simulink model "mdl_foc_platform"  (R2023a)
settings: configuration reference "cfg_FocCodeGeneration_v04" (kept outside this file)
undefined symbols (not defined in the file): Cdbl_nMechSpdPeakVal, cstPermMagTempCoef, cstPolePairNum, cstRefTemp, Gu16_rCtlBrdVltgADCRat_C, Gu16_rGDVltgADCRat_C, Gu16_rPhCurrADCRat_C, Gu16_rSplyVltgADCRat_C, Gu16_tMotoTemp_CUR_ADMotoTempADC_X, Gu16_tPCBTemp_CUR_ADPCBTempADC_X, Gu16_tPwrTubTemp_CUR_ADPwrTubTempADC_X, Gu8_tMotoTemp_CUR, Gu8_tPCBTemp_CUR, Gu8_tPwrTubTemp_CUR, parAmbPermMagFlux, parDirIndc, parPolePairNum, parQdrtIndc
libraries: lib_conversion x10, eeTransforms x1, simulink x1, lib_park_transform x1
(part 1 of 2)
settings Model: DataDictionary=dd_platform_parameter.sldd  EnableAccessToBaseWorkspace=off  PauseTimes=0.1  Creator=WEIFU_YuanXiaoqiang  LastModifiedBy=xiaoqiang.yuan
settings ConfigSetRef: SourceName=cfg_FocCodeGeneration_v04

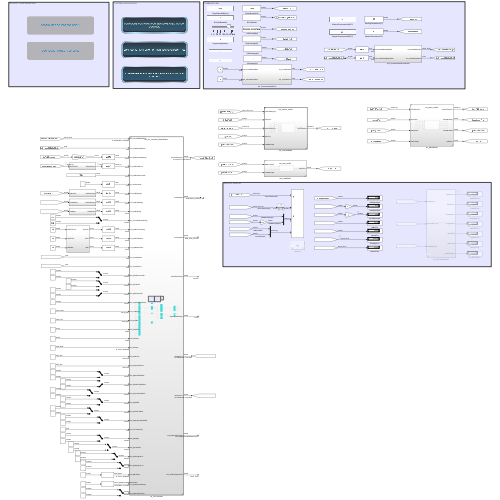
[thumbnail: Simulink's stored preview of the top-level diagram]
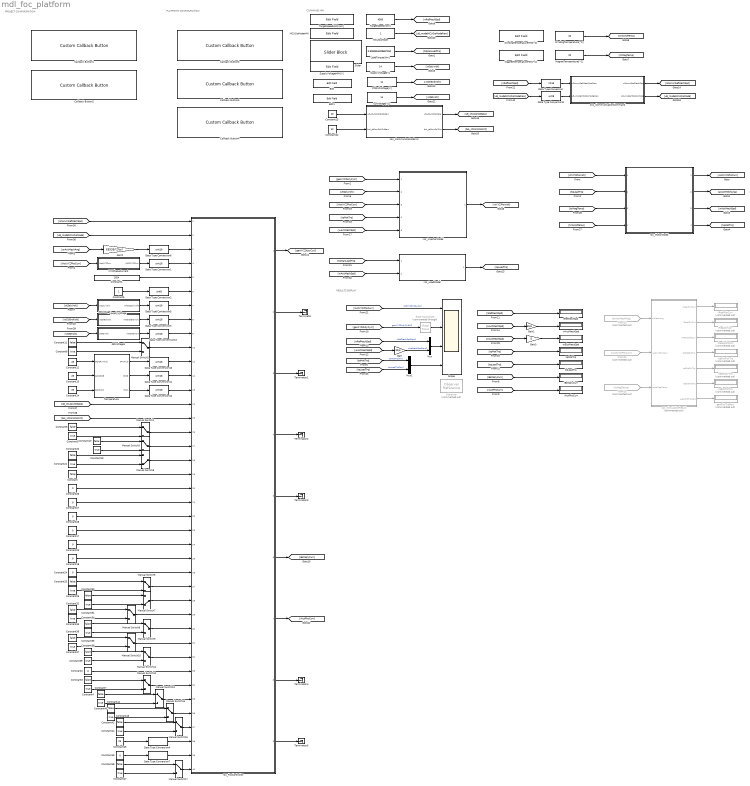
== system mdl_foc_platform ==
  note: PROJECT CONFIGURATION
  note: COMMAND HMI
  note: PLATFORM CONFIGURATION
  note: RESULTS DISPLAY
  Callback Button1 : CustomCallbackButton  Description=BYD 48V Project  Configuration="{\"components\":[{\"name\":\"BackgroundImageComponent\",\"settings\":{\"image\":{\"size\":[0,0],\"src\":\"default\",\"srcOrientation\":\"horizontal\"},\"position\":[0,0,1,1],\"scaleMode\":\"0\"}},{\"name\":\"ButtonStateComponent\",\"settings\":{\"buttonType\":\"momentary\",\"clickFcn\":\"\\nproj = simulinkproject;\\nproj_dir = proj.RootFolder;\\n% configure GEELY\\n%%AST \\nopen_system([proj_dir,'\\\\referenced_model\\\\ASW_AST\\\\ASW_AST.slx']);\\nmodel_path = 'ASW_AST';\\nset_param([model_path,'\\/AST_SlwTask\\/vrs_SysSTM'],...\\n    'LabelModeActiveChoice','GEELY_PROJECT');\\nsave_system([proj_dir,'\\\\referenced_model\\\\ASW_AST\\\\ASW_AST.slx'],'SaveDirtyReferencedModels',true);\\nclose_system([proj_dir,'\\\\referenced_model\\\\ASW_AST\\\\ASW_AST.slx']);\\n\\n%%OBD \\nopen_system([proj_dir,'\\\\referenced_model\\\\ASW_OBD\\\\ASW_OBD.slx']);\\nmodel_path = 'ASW_OBD';\\nset_param([model_path,'\\/OBD_SlwTask\\/rss_ComFaltDia\\/sss_ComFalt\\/ens_HysDeb'],...\\n    'LabelModeActiveChoice','GEELY_PROJECT');\\nset_param([model_path,'\\/OBD_SlwTask\\/rss_FaltResp\\/sss_FaltRespDefd\\/sss_FaltMechSpdRespDefd\\/sss_Else\\/sss_ComFaltMechSpdRespDefd'],...\\n    'LabelModeActiveChoice','GEELY_PROJECT');\\nset_param([model_path,'\\/OBD_SlwTask\\/vrs_FaltEnFlgConf\\/rss_FaltEnFlgConfSenl\\/sss_FaltPrioJudg\\/sss_Else'],...\\n    'LabelModeActiveChoice','GEELY_PROJECT');\\nset_param([model_path,'\\/OBD_SlwTask\\/rss_FaltInfoMng\\/vrs_DSMSaveInfo'],...\\n    'LabelModeActiveChoice','DSMSaveInfoNoNeed');\\nset_param([model_path,'\\/OBD_SlwTask\\/rss_GDVltgLoLvl1Dia\\/sss_GDVltgLoLvl1\\/ens_Deb'],...\\n    'LabelModeActiveChoice','GEELY_PROJECT');\\nset_param([model_path,'\\/OBD_SlwTask\\/rss_GDVltgHiLvl1Dia\\/sss_GDVltgHiLvl1\\/ens_Deb'],...\\n    'LabelModeActiveChoice','GEELY_PROJECT');\\nsave_system([proj_dir,'\\\\referenced_model\\\\ASW_OBD\\\\ASW_OBD.slx'],'SaveDirtyReferencedModels',true);\\nclose_system([proj_dir,'\\\\referenced_model\\\\ASW_OBD\\\\ASW_OBD.slx']);\\n\",\"image\":{\"size\":[180,45],\"srcOrientation\":\"Right\"},\"onValue\":1,\"position\":[0,0,1,1],\"pressDelay\":\"500\",\"pressFcn\":\"\",\"repeatInterval\":\"0\",\"states\":[{\"horizontalAlignment\":\"center\",\"image\":{\"position\":[0.04444444444444445,0.005555555555555536,0.9888888888888889,0.9111111111111111],\"size\":[0.9888888888888889,0.9111111111111111],\"src\":\"data:image\\/svg+xml;base64,PHN2ZyB4bWxucz0iaHR0cDovL3d3dy53My5vcmcvMjAwMC9zdmciIHhtbG5zOnhsaW5rPSJodHRwOi8vd3d3LnczLm9yZy8xOTk5L3hsaW5rIiB2aWV3Qm94PSIwIDAgMTc3LjI1IDQwLjg4Ij48ZGVmcz48c3R5bGU+LmNscy0xe2ZpbGw6dXJsKCNyYWRpYWwtZ3JhZGllbnQpO30uY2xzLTJ7ZmlsbDp1cmwoI2xpbmVhci1ncmFkaWVudCk7fS5jbHMtM3tmaWxsOnVybCgjbGluZWFyLWdyYWRpZW50LTIpO308L3N0eWxlPjxyYWRpYWxHcmFkaWVudCBpZD0icmFkaWFsLWdyYWRpZW50IiBjeD0iOTAuMDkiIGN5PSIyMi42NiIgcj0i ...(+2212 chars)\",\"srcOrientation\":\"Right\"},\"label\":{\"color\":[0,0.4470588235294118,0.7411764705882353],\"icon\":{\"size\":[0,0],\"src\":[],\"srcOrientation\":\"Right\"},\"iconPlacement\":\"left\",\"opacity\":1,\"show\":true,\"text\":{\"content\":\"CONFIGURE PROJECT FOR GEELY\",\"font\":\"Helvetica\",\"fontSize\":4.2}},\"labelOffset\":[0,0],\"verticalAlignment\":\"middle\"},{\"horizontalAlignment\":\"center\",\"image\":{\"position\":[0.04444444444444445,0.005555555555555536,0.9888888888888889,0.9111111111111111],\"size\":[0.9888888888888889,0.9111111111111111],\"src\":\"data:image\\/svg+xml;base64,PHN2ZyB4bWxucz0iaHR0cDovL3d3dy53My5vcmcvMjAwMC9zdmciIHhtbG5zOnhsaW5rPSJodHRwOi8vd3d3LnczLm9yZy8xOTk5L3hsaW5rIiB2aWV3Qm94PSIwIDAgMTc3LjI1IDQwLjg4Ij48ZGVmcz48c3R5bGU+LmNscy0xe2ZpbGw6dXJsKCNyYWRpYWwtZ3JhZGllbnQpO30uY2xzLTJ7ZmlsbDp1cmwoI2xpbmVhci1ncmFkaWVudCk7fS5jbHMtM3tmaWxsOnVybCgjbGluZWFyLWdyYWRpZW50LTIpO308L3N0eWxlPjxyYWRpYWxHcmFkaWVudCBpZD0icmFkaWFsLWdyYWRpZW50IiBjeD0iOTAuMDkiIGN5PSIyMi42NiIgcj0i ...(+2216 chars)\",\"srcOrientation\":\"Right\"},\"label\":{\"color\":[1,1,0.78,1],\"icon\":{\"size\":[0,0],\"src\":[],\"srcOrientation\":\"Right\"},\"iconPlacement\":\"left\",\"opacity\":1,\"show\":true,\"text\":{\"content\":\"CONFIGURE PROJECT FOR GEELY\",\"font\":\"Helvetica\",\"fontSize\":4.2}},\"labelOffset\":[0.025,0],\"verticalAlignment\":\"middle\"},{\"horizontalAlignment\":\"center\",\"image\":{\"position\":[0.04444444444444445,0.005555555555555536,0.9888888888888889,0.9111111111111111],\"size\":[0.9888888888888889,0.9111111111111111],\"src\":\"data:image\\/svg+xml;base64,PHN2ZyB4bWxucz0iaHR0cDovL3d3dy53My5vcmcvMjAwMC9zdmciIHhtbG5zOnhsaW5rPSJodHRwOi8vd3d3LnczLm9yZy8xOTk5L3hsaW5rIiB2aWV3Qm94PSIwIDAgMTc3LjI1IDQwLjg4Ij48ZGVmcz48c3R5bGU+LmNscy0xe2ZpbGw6dXJsKCNyYWRpYWwtZ3JhZGllbnQpO30uY2xzLTJ7ZmlsbDp1cmwoI2xpbmVhci1ncmFkaWVudCk7fS5jbHMtM3tmaWxsOnVybCgjbGluZWFyLWdyYWRpZW50LTIpO308L3N0eWxlPjxyYWRpYWxHcmFkaWVudCBpZD0icmFkaWFsLWdyYWRpZW50IiBjeD0iOTAuMDkiIGN5PSIyMi42NiIgcj0i ...(+2212 chars)\",\"srcOrientation\":\"Right\"},\"label\":{\"color\":[1,1,0.78,1],\"icon\":{\"size\":[0,0],\"src\":[],\"srcOrientation\":\"Right\"},\"iconPlacement\":\"left\",\"opacity\":1,\"show\":true,\"text\":{\"content\":\"CONFIGURE PROJECT FOR GEELY\",\"font\":\"Helvetica\",\"fontSize\":4.2}},\"labelOffset\":[0,0],\"verticalAlignment\":\"middle\"},{\"horizontalAlignment\":\"center\",\"image\":{\"position\":[0.04444444444444445,0.005555555555555536,0.9888888888888889,0.9111111111111111],\"size\":[0.9888888888888889,0.9111111111111111],\"src\":\"data:image\\/svg+xml;base64,PHN2ZyB4bWxucz0iaHR0cDovL3d3dy53My5vcmcvMjAwMC9zdmciIHhtbG5zOnhsaW5rPSJodHRwOi8vd3d3LnczLm9yZy8xOTk5L3hsaW5rIiB2aWV3Qm94PSIwIDAgMTc3LjI1IDQwLjg4Ij48ZGVmcz48c3R5bGU+LmNscy0xe2ZpbGw6dXJsKCNyYWRpYWwtZ3JhZGllbnQpO30uY2xzLTJ7ZmlsbDp1cmwoI2xpbmVhci1ncmFkaWVudCk7fS5jbHMtM3tmaWxsOnVybCgjbGluZWFyLWdyYWRpZW50LTIpO308L3N0eWxlPjxyYWRpYWxHcmFkaWVudCBpZD0icmFkaWFsLWdyYWRpZW50IiBjeD0iOTAuMDkiIGN5PSIyMi42NiIgcj0i ...(+2216 chars)\",\"srcOrientation\":\"Right\"},\"label\":{\"color\":[1,1,0.78,1],\"icon\":{\"size\":[0,0],\"src\":[],\"srcOrientation\":\"Right\"},\"iconPlacement\":\"left\",\"opacity\":1,\"show\":true,\"text\":{\"content\":\"CONFIGURE PROJECT FOR GEELY\",\"font\":\"Helvetica\",\"fontSize\":4.2}},\"labelOffset\":[0.025,0],\"verticalAlignment\":\"middle\"}]}},{\"name\":\"ForegroundImageComponent\",\"settings\":{\"image\":{\"size\":[0,0],\"src\":\"default\",\"srcOrientation\":\"horizontal\"},\"isForeground\":1,\"position\":[0,0,1,1],\"scaleMode\":\"0\"}}],\"settings\":{\"BindingType\":\"param\",\"aspectRatio\":3.7777777777777777,\"backgroundColor\":[255,255,255,\"1\"],\"backgroundOffset\":0.5,\"backgroundOpacity\":1,\"fixedAspectRatio\":\"off\",\"foregroundColor\":[252,252,196],\"showBackgroundColor\":false,\"variant\":\"callback\",\"version\":\"R2022b\"},\"type\":\"Button\"}"  CustomBackgroundColor="{\"color\":[0.6509803921568628,0.6509803921568628,0.6509803921568628],\"show\":true}"
  Callback Button2 : CustomCallbackButton  Description=BYD 48V Project  Configuration="{\"components\":[{\"name\":\"BackgroundImageComponent\",\"settings\":{\"image\":{\"size\":[0,0],\"src\":\"default\",\"srcOrientation\":\"horizontal\"},\"position\":[0,0,1,1],\"scaleMode\":\"0\"}},{\"name\":\"ButtonStateComponent\",\"settings\":{\"buttonType\":\"momentary\",\"clickFcn\":\"\\nproj = simulinkproject;\\nproj_dir = proj.RootFolder;\\n% configure CRRC\\n%%AST \\nopen_system([proj_dir,'\\\\referenced_model\\\\ASW_AST\\\\ASW_AST.slx']);\\nmodel_path = 'ASW_AST';\\nset_param([model_path,'\\/AST_SlwTask\\/vrs_SysSTM'],...\\n    'LabelModeActiveChoice','CRRC_PROJECT');\\nsave_system([proj_dir,'\\\\referenced_model\\\\ASW_AST\\\\ASW_AST.slx'],'SaveDirtyReferencedModels',true);\\nclose_system([proj_dir,'\\\\referenced_model\\\\ASW_AST\\\\ASW_AST.slx']);\\n\\n%%OBD \\nopen_system([proj_dir,'\\\\referenced_model\\\\ASW_OBD\\\\ASW_OBD.slx']);\\nmodel_path = 'ASW_OBD';\\nset_param([model_path,'\\/OBD_SlwTask\\/rss_ComFaltDia\\/sss_ComFalt\\/ens_HysDeb'],...\\n    'LabelModeActiveChoice','CRRC_PROJECT');\\nset_param([model_path,'\\/OBD_SlwTask\\/rss_FaltResp\\/sss_FaltRespDefd\\/sss_FaltMechSpdRespDefd\\/sss_Else\\/sss_ComFaltMechSpdRespDefd'],...\\n    'LabelModeActiveChoice','CRRC_PROJECT');\\nset_param([model_path,'\\/OBD_SlwTask\\/vrs_FaltEnFlgConf\\/rss_FaltEnFlgConfSenl\\/sss_FaltPrioJudg\\/sss_Else'],...\\n    'LabelModeActiveChoice','CRRC_PROJECT');\\nset_param([model_path,'\\/OBD_SlwTask\\/rss_FaltInfoMng\\/vrs_DSMSaveInfo'],...\\n    'LabelModeActiveChoice','DSMSaveInfoNeed');\\nset_param([model_path,'\\/OBD_SlwTask\\/rss_GDVltgLoLvl1Dia\\/sss_GDVltgLoLvl1\\/ens_Deb'],...\\n    'LabelModeActiveChoice','CRRC_PROJECT');\\nset_param([model_path,'\\/OBD_SlwTask\\/rss_GDVltgHiLvl1Dia\\/sss_GDVltgHiLvl1\\/ens_Deb'],...\\n    'LabelModeActiveChoice','CRRC_PROJECT');\\nsave_system([proj_dir,'\\\\referenced_model\\\\ASW_OBD\\\\ASW_OBD.slx'],'SaveDirtyReferencedModels',true);\\nclose_system([proj_dir,'\\\\referenced_model\\\\ASW_OBD\\\\ASW_OBD.slx']);\\n\",\"image\":{\"size\":[180,45],\"srcOrientation\":\"Right\"},\"onValue\":1,\"position\":[0,0,1,1],\"pressDelay\":\"500\",\"pressFcn\":\"\",\"repeatInterval\":\"0\",\"states\":[{\"horizontalAlignment\":\"center\",\"image\":{\"position\":[0.04444444444444445,0.005555555555555536,0.9888888888888889,0.9111111111111111],\"size\":[0.9888888888888889,0.9111111111111111],\"src\":\"data:image\\/svg+xml;base64,PHN2ZyB4bWxucz0iaHR0cDovL3d3dy53My5vcmcvMjAwMC9zdmciIHhtbG5zOnhsaW5rPSJodHRwOi8vd3d3LnczLm9yZy8xOTk5L3hsaW5rIiB2aWV3Qm94PSIwIDAgMTc3LjI1IDQwLjg4Ij48ZGVmcz48c3R5bGU+LmNscy0xe2ZpbGw6dXJsKCNyYWRpYWwtZ3JhZGllbnQpO30uY2xzLTJ7ZmlsbDp1cmwoI2xpbmVhci1ncmFkaWVudCk7fS5jbHMtM3tmaWxsOnVybCgjbGluZWFyLWdyYWRpZW50LTIpO308L3N0eWxlPjxyYWRpYWxHcmFkaWVudCBpZD0icmFkaWFsLWdyYWRpZW50IiBjeD0iOTAuMDkiIGN5PSIyMi42NiIgcj0i ...(+2212 chars)\",\"srcOrientation\":\"Right\"},\"label\":{\"color\":[0,0.4470588235294118,0.7411764705882353],\"icon\":{\"size\":[0,0],\"src\":[],\"srcOrientation\":\"Right\"},\"iconPlacement\":\"left\",\"opacity\":1,\"show\":true,\"text\":{\"content\":\"CONFIGURE PROJECT FOR CRRC\",\"font\":\"Helvetica\",\"fontSize\":4.2}},\"labelOffset\":[0,0],\"verticalAlignment\":\"middle\"},{\"horizontalAlignment\":\"center\",\"image\":{\"position\":[0.04444444444444445,0.005555555555555536,0.9888888888888889,0.9111111111111111],\"size\":[0.9888888888888889,0.9111111111111111],\"src\":\"data:image\\/svg+xml;base64,PHN2ZyB4bWxucz0iaHR0cDovL3d3dy53My5vcmcvMjAwMC9zdmciIHhtbG5zOnhsaW5rPSJodHRwOi8vd3d3LnczLm9yZy8xOTk5L3hsaW5rIiB2aWV3Qm94PSIwIDAgMTc3LjI1IDQwLjg4Ij48ZGVmcz48c3R5bGU+LmNscy0xe2ZpbGw6dXJsKCNyYWRpYWwtZ3JhZGllbnQpO30uY2xzLTJ7ZmlsbDp1cmwoI2xpbmVhci1ncmFkaWVudCk7fS5jbHMtM3tmaWxsOnVybCgjbGluZWFyLWdyYWRpZW50LTIpO308L3N0eWxlPjxyYWRpYWxHcmFkaWVudCBpZD0icmFkaWFsLWdyYWRpZW50IiBjeD0iOTAuMDkiIGN5PSIyMi42NiIgcj0i ...(+2216 chars)\",\"srcOrientation\":\"Right\"},\"label\":{\"color\":[1,1,0.78,1],\"icon\":{\"size\":[0,0],\"src\":[],\"srcOrientation\":\"Right\"},\"iconPlacement\":\"left\",\"opacity\":1,\"show\":true,\"text\":{\"content\":\"CONFIGURE PROJECT FOR CRRC\",\"font\":\"Helvetica\",\"fontSize\":4.2}},\"labelOffset\":[0.025,0],\"verticalAlignment\":\"middle\"},{\"horizontalAlignment\":\"center\",\"image\":{\"position\":[0.04444444444444445,0.005555555555555536,0.9888888888888889,0.9111111111111111],\"size\":[0.9888888888888889,0.9111111111111111],\"src\":\"data:image\\/svg+xml;base64,PHN2ZyB4bWxucz0iaHR0cDovL3d3dy53My5vcmcvMjAwMC9zdmciIHhtbG5zOnhsaW5rPSJodHRwOi8vd3d3LnczLm9yZy8xOTk5L3hsaW5rIiB2aWV3Qm94PSIwIDAgMTc3LjI1IDQwLjg4Ij48ZGVmcz48c3R5bGU+LmNscy0xe2ZpbGw6dXJsKCNyYWRpYWwtZ3JhZGllbnQpO30uY2xzLTJ7ZmlsbDp1cmwoI2xpbmVhci1ncmFkaWVudCk7fS5jbHMtM3tmaWxsOnVybCgjbGluZWFyLWdyYWRpZW50LTIpO308L3N0eWxlPjxyYWRpYWxHcmFkaWVudCBpZD0icmFkaWFsLWdyYWRpZW50IiBjeD0iOTAuMDkiIGN5PSIyMi42NiIgcj0i ...(+2212 chars)\",\"srcOrientation\":\"Right\"},\"label\":{\"color\":[1,1,0.78,1],\"icon\":{\"size\":[0,0],\"src\":[],\"srcOrientation\":\"Right\"},\"iconPlacement\":\"left\",\"opacity\":1,\"show\":true,\"text\":{\"content\":\"CONFIGURE PROJECT FOR CRRC\",\"font\":\"Helvetica\",\"fontSize\":4.2}},\"labelOffset\":[0,0],\"verticalAlignment\":\"middle\"},{\"horizontalAlignment\":\"center\",\"image\":{\"position\":[0.04444444444444445,0.005555555555555536,0.9888888888888889,0.9111111111111111],\"size\":[0.9888888888888889,0.9111111111111111],\"src\":\"data:image\\/svg+xml;base64,PHN2ZyB4bWxucz0iaHR0cDovL3d3dy53My5vcmcvMjAwMC9zdmciIHhtbG5zOnhsaW5rPSJodHRwOi8vd3d3LnczLm9yZy8xOTk5L3hsaW5rIiB2aWV3Qm94PSIwIDAgMTc3LjI1IDQwLjg4Ij48ZGVmcz48c3R5bGU+LmNscy0xe2ZpbGw6dXJsKCNyYWRpYWwtZ3JhZGllbnQpO30uY2xzLTJ7ZmlsbDp1cmwoI2xpbmVhci1ncmFkaWVudCk7fS5jbHMtM3tmaWxsOnVybCgjbGluZWFyLWdyYWRpZW50LTIpO308L3N0eWxlPjxyYWRpYWxHcmFkaWVudCBpZD0icmFkaWFsLWdyYWRpZW50IiBjeD0iOTAuMDkiIGN5PSIyMi42NiIgcj0i ...(+2216 chars)\",\"srcOrientation\":\"Right\"},\"label\":{\"color\":[1,1,0.78,1],\"icon\":{\"size\":[0,0],\"src\":[],\"srcOrientation\":\"Right\"},\"iconPlacement\":\"left\",\"opacity\":1,\"show\":true,\"text\":{\"content\":\"CONFIGURE PROJECT FOR CRRC\",\"font\":\"Helvetica\",\"fontSize\":4.2}},\"labelOffset\":[0.025,0],\"verticalAlignment\":\"middle\"}]}},{\"name\":\"ForegroundImageComponent\",\"settings\":{\"image\":{\"size\":[0,0],\"src\":\"default\",\"srcOrientation\":\"horizontal\"},\"isForeground\":1,\"position\":[0,0,1,1],\"scaleMode\":\"0\"}}],\"settings\":{\"BindingType\":\"param\",\"aspectRatio\":3.7777777777777777,\"backgroundColor\":[255,255,255,\"1\"],\"backgroundOffset\":0.5,\"backgroundOpacity\":1,\"fixedAspectRatio\":\"off\",\"foregroundColor\":[252,252,196],\"showBackgroundColor\":false,\"variant\":\"callback\",\"version\":\"R2022b\"},\"type\":\"Button\"}"  CustomBackgroundColor="{\"color\":[0.6509803921568628,0.6509803921568628,0.6509803921568628],\"show\":true}"
  Callback Button3 : CustomCallbackButton  Configuration="{\"components\":[{\"name\":\"BackgroundImageComponent\",\"settings\":{\"image\":{\"size\":[0,0],\"src\":\"default\",\"srcOrientation\":\"horizontal\"},\"position\":[0,0,1,1],\"scaleMode\":\"0\"}},{\"name\":\"ButtonStateComponent\",\"settings\":{\"buttonType\":\"momentary\",\"clickFcn\":\"\\nsave_system;\\n\\nproj = simulinkproject;\\nproj_dir = proj.RootFolder;\\nconfiguration_dd = Simulink.data.dictionary.open([proj_dir,'\\\\data_dictionary\\\\dd_foc_configuration_parameter.sldd']);\\ninterface_dd = Simulink.data.dictionary.open([proj_dir,'\\\\data_dictionary\\\\dd_foc_data_type.sldd']);\\nconfiguration_data_obj = getSection(configuration_dd,'Design Data');\\ninterface_data_obj = getSection(interface_dd,'Design Data');\\n\\n% configure motor control components\\n    %Fast task\\nopen_system([proj_dir,'\\\\referenced_model\\\\ASW_DcycGen\\\\ASW_DcycGen.slx']);\\nmodel_path = 'ASW_DcycGen';\\nset_param([model_path,'\\/DcycGen_FstTask\\/vrs_ModulElecAgCalc'],...\\n    'LabelModeActiveChoice','cstSensCtrlLbl');\\nset_param([model_path,'\\/DcycGen_FstTask\\/vrs_FstTaskIn'],...\\n    'LabelModeActiveChoice','cstSensCtrlLbl');\\nset_param([model_path,'\\/DcycGen_FstTask\\/vrs_FstTaskOut'],...\\n    'LabelModeActiveChoice','cstSensCtrlLbl');\\n\\nsave_system([proj_dir,'\\\\referenced_model\\\\ASW_DcycGen\\\\ASW_DcycGen.slx'],'SaveDirtyReferencedModels',true);\\nclose_system([proj_dir,'\\\\referenced_model\\\\ASW_DcycGen\\\\ASW_DcycGen.slx']);\\n\\nconfigBus_obj = getValue(getEntry(configuration_data_obj,'BUS_DCYCGEN_FST_TASK_IN_SENSVRNT'));\\nbus_entry = getEntry(interface_data_obj,'BUS_DCYCGEN_FST_TASK_IN');\\nnewbus_obj = getValue(bus_entry);\\nnewbus_obj.Elements = configBus_obj.Elements;\\nsetValue(bus_entry,newbus_obj);\\n\\nconfigBus_obj = getValue(getEntry(configuration_data_obj,'BUS_DCYCGEN_FST_TASK_OUT_SENSVRNT'));\\nbus_entry = getEntry(interface_data_obj,'BUS_DCYCGEN_FST_TASK_OUT');\\nnewbus_obj = getValue(bus_entry);\\nnewbus_obj.Elements = configBus_obj.Elements;\\nsetValue(bus_entry,newbus_obj);\\n\\n    %Medium task\\nopen_system([proj_dir,'\\\\referenced_model\\\\ASW_PhVltgGen\\\\ASW_PhVltgGen.slx']);\\nmodel_path = 'ASW_PhVltgGen';\\nset_param([model_path,'\\/PhVltgGen_MedTask\\/vrs_ActElecAgElecSpdCmpt'],...\\n    'LabelModeActiveChoice','cstSensCtrlLbl');  \\nset_param([model_path,'\\/PhVltgGen_MedTask\\/vrs_ParkTrasf'],...\\n    'LabelModeActiveChoice','cstSensCtrlLbl'); \\nset_param([model_path,'\\/PhVltgGen_MedTask\\/vrs_CurrCtl'],...\\n    'LabelModeActiveChoice','cstSensCtrlLbl'); \\nset_param([model_path,'\\/PhVltgGen_MedTask\\/vrs_StrtUpElecAgCalc'],...\\n    'LabelModeActiveChoice','cstSensCtrlLbl'); \\nset_param([model_path,'\\/PhVltgGen_MedTask\\/vrs_MedTaskIn'],...\\n    'LabelModeActiveChoice','cstSensCtrlLbl');\\nset_param([model_path,'\\/PhVltgGen_MedTask\\/vrs_MedTaskOut'],...\\n    'LabelModeActiveChoice','cstSensCtrlLbl');\\n\\nsave_system([proj_dir,'\\\\referenced_model\\\\ASW_PhVltgGen\\\\ASW_PhVltgGen.slx'],'SaveDirtyReferencedModels',true);\\nclose_system([proj_dir,'\\\\referenced_model\\\\ASW_PhVltgGen\\\\ASW_PhVltgGen.slx']);\\n\\nconfigBus_obj = getValue(getEntry(configuration_data_obj,'BUS_PHVLTGGEN_MED_TASK_IN_SENSVRNT'));\\nbus_entry = getEntry(interface_data_obj,'BUS_PHVLTGGEN_MED_TASK_IN');\\nnewbus_obj = getValue(bus_entry);\\nnewbus_obj.Elements = configBus_obj.Elements;\\nsetValue(bus_entry,newbus_obj);\\n\\nconfigBus_obj = getValue(getEntry(configuration_data_obj,'BUS_PHVLTGGEN_MED_TASK_OUT_SENSVRNT'));\\nbus_entry = getEntry(interface_data_obj,'BUS_PHVLTGGEN_MED_TASK_OUT');\\nnewbus_obj = getValue(bus_entry);\\nnewbus_obj.Elements = configBus_obj.Elements;\\nsetValue(bus_entry,newbus_obj);\\n\\n    %Slow task\\nopen_system([proj_dir,'\\\\referenced_model\\\\ASW_PhCurrGen\\\\ASW_PhCurrGen.slx']);\\nmodel_path = 'ASW_PhCurrGen';\\nset_param([model_path,'\\/PhCurrGen_SlwTask\\/vrs_MotoSTM'],...\\n    'LabelModeActiveChoice','cstSensCtrlLbl');\\nset_param([model_path,'\\/PhCurrGen_SlwTask\\/vrs_StrtUpPrcdChk'],...\\n    'LabelModeActiveChoice','cstSensCtrlLbl'); \\nset_param([model_path,'\\/PhCurrGen_SlwTask\\/vrs_StrtUpRefTqCalc'],...\\n    'LabelModeActiveChoice','cstSensCtrlLbl'); \\nset_param([model_path,'\\/PhCurrGen_SlwTask\\/vrs_ElecSpdCtl'],...\\n    'LabelModeActiveChoice','cstSensCtrlLbl');\\nset_param([model_path,'\\/PhCurrGen_SlwTask\\/vrs_SlwTaskIn'],...\\n    'LabelModeActiveChoice','cstSensCtrlLbl');  \\nset_param([model_path,'\\/PhCurrGen_SlwTask\\/vrs_SlwTaskOut'],...\\n    'LabelModeActiveChoice','cstSensCtrlLbl');    \\nsave_system([proj_dir,'\\\\referenced_model\\\\ASW_PhCurrGen\\\\ASW_PhCurrGen.slx'],'SaveDirtyReferencedModels',true);\\nclose_system([proj_dir,'\\\\referenced_model\\\\ASW_PhCurrGen\\\\ASW_PhCurrGen.slx']);\\n\\nconfigBus_obj = getValue(getEntry(configuration_data_obj,'BUS_PHCURRGEN_SLW_TASK_IN_SENSVRNT'));\\nbus_entry = getEntry(interface_data_obj,'BUS_PHCURRGEN_SLW_TASK_IN');\\nnewbus_obj = getValue(bus_entry);\\nnewbus_obj.Elements = configBus_obj.Elements;\\nsetValue(bus_entry,newbus_obj);\\n\\nconfigBus_obj = getValue(getEntry(configuration_data_obj,'BUS_PHCURRGEN_SLW_TASK_OUT_SENSVRNT'));\\nbus_entry = getEntry(interface_data_obj,'BUS_PHCURRGEN_SLW_TASK_OUT');\\nnewbus_obj = getValue(bus_entry);\\nnewbus_obj.Elements = configBus_obj.Elements;\\nsetValue(bus_entry,newbus_obj);\\n\\n% configure assistant components\\nopen_system([proj_dir,'\\\\referenced_model\\\\ASW_AST\\\\ASW_AST.slx']);\\nmodel_path = 'ASW_AST';\\nset_param([model_path,'\\/AST_SlwTask\\/vrs_SensAgCalib'],...\\n    'LabelModeActiveChoice','cstSensCtrlLbl');\\nset_param([model_path,'\\/AST_SlwTask\\/vrs_RefElecSpdCalc'],...\\n    'LabelModeActiveChoice','cstSensCtrlLbl');\\nset_param([model_path,'\\/AST_SlwTask\\/vrs_ShOffFlgConf'],...\\n    'LabelModeActiveChoice','cstSensCtrlLbl');\\nset_param([model_path,'\\/AST_SlwTask\\/vrs_AgEvalModeCalc'],...\\n    'LabelModeActiveChoice','cstSensCtrlLbl');\\nset_param([model_path,'\\/AST_SlwTask\\/vrs_SlwTaskIn'],...\\n    'LabelModeActiveChoice','cstSensCtrlLbl');\\nset_param([model_path,'\\/AST_SlwTask\\/vrs_SlwTaskOut'],...\\n    'LabelModeActiveChoice','cstSensCtrlLbl');\\nsave_system([proj_dir,'\\\\referenced_model\\\\ASW_AST\\\\ASW_AST.slx'],'SaveDirtyReferencedModels',true);\\nclose_system([proj_dir,'\\\\referenced_model\\\\ASW_AST\\\\ASW_AST.slx']);\\n\\nconfigBus_obj = getValue(getEntry(configuration_data_obj,'BUS_AST_SLW_TASK_IN_SENSVRNT'));\\nbus_entry = getEntry(interface_data_obj,'BUS_AST_SLW_TASK_IN');\\nnewbus_obj = getValue(bus_entry);\\nnewbus_obj.Elements = configBus_obj.Elements;\\nsetValue(bus_entry,newbus_obj);\\n\\nconfigBus_obj = getValue(getEntry(configuration_data_obj,'BUS_AST_SLW_TASK_OUT_SENSVRNT'));\\nbus_entry = getEntry(interface_data_obj,'BUS_AST_SLW_TASK_OUT');\\nnewbus_obj = getValue(bus_entry);\\nnewbus_obj.Elements = configBus_obj.Elements;\\nsetValue(bus_entry,newbus_obj);\\n\\n% configure OBD components\\nopen_system([proj_dir,'\\\\referenced_model\\\\ASW_OBD\\\\ASW_OBD.slx']);\\nmodel_path = 'ASW_OBD';\\nset_param([model_path,'\\/OBD_SlwTask\\/vrs_MotoStallDia'],...\\n    'LabelModeActiveChoice','cstSensCtrlLbl');\\nset_param([model_path,'\\/OBD_SlwTask\\/vrs_FaltEnFlgConf'],...\\n    'LabelModeActiveChoice','cstSensCtrlLbl');\\nset_param([model_path,'\\/OBD_SlwTask\\/vrs_PhiSensFaltDia'],...\\n    'LabelModeActiveChoice','cstSensCtrlLbl');\\nset_param([model_path,'\\/OBD_SlwTask\\/vrs_SlwTaskIn'],...\\n    'LabelModeActiveChoice','cstSensCtrlLbl');\\nset_param([model_path,'\\/OBD_SlwTask\\/vrs_SlwTaskOut'],...\\n    'LabelModeActiveChoice','cstSensCtrlLbl');\\nsave_system([proj_dir,'\\\\referenced_model\\\\ASW_OBD\\\\ASW_OBD.slx'],'SaveDirtyReferencedModels',true);\\nclose_system([proj_dir,'\\\\referenced_model\\\\ASW_OBD\\\\ASW_OBD.slx']);\\n\\nconfigBus_obj = getValue(getEntry(configuration_data_obj,'BUS_OBD_SLW_TASK_OUT_SENSVRNT'));\\nbus_entry = getEntry(interface_data_obj,'BUS_OBD_SLW_TASK_OUT');\\nnewbus_obj = getValue(bus_entry);\\nnewbus_obj.Elements = configBus_obj.Elements;\\nsetValue(bus_entry,newbus_obj);\\n\\nconfigBus_obj = getValue(getEntry(configuration_data_obj,'BUS_OBD_SLW_TASK_IN_SENSVRNT'));\\nbus_entry = getEntry(interface_data_obj,'BUS_OBD_SLW_TASK_IN');\\nnewbus_obj = getValue(bus_entry);\\nnewbus_obj.Elements = configBus_obj.Elements;\\nsetValue(bus_entry,newbus_obj);\\n\\n% configure SigIn componets\\nopen_system([proj_dir,'\\\\referenced_model\\\\ASW_SigIn\\\\ASW_SigIn.slx']);\\nmodel_path = 'ASW_SigIn';\\n    %Medium task\\nset_param([model_path,'\\/SigIn_MedTask\\/vrs_ElecAgCalc'],...\\n    'LabelModeActiveChoice','cstSensCtrlLbl');\\nset_param([model_path,'\\/SigIn_MedTask\\/vrs_MedTaskIn'],...\\n    'LabelModeActiveChoice','cstSensCtrlLbl');\\nset_param([model_path,'\\/SigIn_MedTask\\/vrs_MedTaskOut'],...\\n    'LabelModeActiveChoice','cstSensCtrlLbl');\\n    %Slow task\\nset_param([model_path,'\\/SigIn_SlwTask\\/vrs_SlwTaskOut'],...\\n    'LabelModeActiveChoice','cstSensCtrlLbl');\\nsave_system([proj_dir,'\\\\referenced_model\\\\ASW_SigIn\\\\ASW_SigIn.slx'],'SaveDirtyReferencedModels',true);\\nclose_system([proj_dir,'\\\\referenced_model\\\\ASW_SigIn\\\\ASW_SigIn.slx']);\\n\\nconfigBus_obj = getValue(getEntry(configuration_data_obj,'BUS_SIGIN_MED_TASK_IN_SENSVRNT'));\\nbus_entry = getEntry(interface_data_obj,'BUS_SIGIN_MED_TASK_IN');\\nnewbus_obj = getValue(bus_entry);\\nnewbus_obj.Elements = configBus_obj.Elements;\\nsetValue(bus_entry,newbus_obj);\\n\\nconfigBus_obj = getValue(getEntry(configuration_data_obj,'BUS_SIGIN_MED_TASK_OUT_SENSVRNT'));\\nbus_entry = getEntry(interface_data_obj,'BUS_SIGIN_MED_TASK_OUT');\\nnewbus_obj = getValue(bus_entry);\\nnewbus_obj.Elements = configBus_obj.Elements;\\nsetValue(bus_entry,newbus_obj);\\n\\nconfigBus_obj = getValue(getEntry(configuration_data_obj,'BUS_SIGIN_SLW_TASK_OUT_SENSVRNT'));\\nbus_entry = getEntry(interface_data_obj,'BUS_SIGIN_SLW_TASK_OUT');\\nnewbus_obj = getValue(bus_entry);\\nnewbus_obj.Elements = configBus_obj.Elements;\\nsetValue(bus_entry,newbus_obj);\\n\\n% configure interfaces of FOC platform\\nopen_system([proj_dir,'\\\\referenced_subsystem\\\\rss_foc_controller_NewPlatform.slx']);\\nmodel_path = 'rss_foc_controller_NewPlatform';\\nset_param([model_path,'\\/vrs_DcycGenFstTaskIn'],'LabelModeActiveChoice','cstSensCtrlLbl');\\nset_param([model_path,'\\/vrs_DcycGenFstTaskOut'],'LabelModeActiveChoice','cstSensCtrlLbl');\\nset_param([model_path,'\\/vrs_PhVltgGenMedTaskIn'],'LabelModeActiveChoice','cstSensCtrlLbl');\\nset_param([model_path,'\\/vrs_PhVltgGenMedTaskOut'],'LabelModeActiveChoice','cstSensCtrlLbl');\\nset_param([model_path,'\\/vrs_PhCurrGenSlwTaskIn'],'LabelModeActiveChoice','cstSensCtrlLbl');\\nset_param([model_path,'\\/vrs_PhCurrGenSlwTaskOut'],'LabelModeActiveChoice','cstSensCtrlLbl');\\nset_param([model_path,'\\/vrs_ASTSlwTaskIn'],'LabelModeActiveChoice','cstSensCtrlLbl');\\nset_param([model_path,'\\/vrs_ASTSlwTaskOut'],'LabelModeActiveChoice','cstSensCtrlLbl');\\nset_param([model_path,'\\/vrs_OBDSlwTaskIn'],'LabelModeActiveChoice','cstSensCtrlLbl');\\nset_param([model_path,'\\/vrs_OBDSlwTaskOut'],'LabelModeActiveChoice','cstSensCtrlLbl');\\nset_param([model_path,'\\/vrs_SigInMedTaskIn'],'LabelModeActiveChoice','cstSensCtrlLbl');\\nset_param([model_path,'\\/vrs_SigInMedTaskOut'],'LabelModeActiveChoice','cstSensCtrlLbl');\\nset_param([model_path,'\\/vrs_SigInSlwTaskOut'],'LabelModeActiveChoice','cstSensCtrlLbl');\\nsave_system([proj_dir,'\\\\referenced_subsystem\\\\rss_foc_controller_NewPlatform.slx'],'SaveDirtyReferencedModels',true);\\nclose_system([proj_dir,'\\\\referenced_subsystem\\\\rss_foc_controller_NewPlatform.slx']);\\n\",\"image\":{\"size\":[180,45],\"srcOrientation\":\"Right\"},\"onValue\":1,\"position\":[0,0,1,1],\"pressDelay\":\"500\",\"pressFcn\":\"\",\"repeatInterval\":\"0\",\"states\":[{\"horizontalAlignment\":\"center\",\"image\":{\"position\":[0.04444444444444445,0.005555555555555536,0.9888888888888889,0.9111111111111111],\"size\":[0.9888888888888889,0.9111111111111111],\"src\":\"data:image\\/svg+xml;base64,PHN2ZyB4bWxucz0iaHR0cDovL3d3dy53My5vcmcvMjAwMC9zdmciIHhtbG5zOnhsaW5rPSJodHRwOi8vd3d3LnczLm9yZy8xOTk5L3hsaW5rIiB2aWV3Qm94PSIwIDAgMTc3LjI1IDQwLjg4Ij48ZGVmcz48c3R5bGU+LmNscy0xe2ZpbGw6dXJsKCNyYWRpYWwtZ3JhZGllbnQpO30uY2xzLTJ7ZmlsbDp1cmwoI2xpbmVhci1ncmFkaWVudCk7fS5jbHMtM3tmaWxsOnVybCgjbGluZWFyLWdyYWRpZW50LTIpO308L3N0eWxlPjxyYWRpYWxHcmFkaWVudCBpZD0icmFkaWFsLWdyYWRpZW50IiBjeD0iOTAuMDkiIGN5PSIyMi42NiIgcj0i ...(+2212 chars)\",\"srcOrientation\":\"Right\"},\"label\":{\"color\":[1,1,0.78,1],\"icon\":{\"size\":[0,0],\"src\":[],\"srcOrientation\":\"Right\"},\"iconPlacement\":\"left\",\"opacity\":1,\"show\":true,\"text\":{\"content\":\"CONFIGURE PLATFORM FOR SENSOR-BASED MOTOR CONTROL\",\"font\":\"Helvetica\",\"fontSize\":2.375646}},\"labelOffset\":[0,0],\"verticalAlignment\":\"middle\"},{\"horizontalAlignment\":\"center\",\"image\":{\"position\":[0.04444444444444445,0.005555555555555536,0.9888888888888889,0.9111111111111111],\"size\":[0.9888888888888889,0.9111111111111111],\"src\":\"data:image\\/svg+xml;base64,PHN2ZyB4bWxucz0iaHR0cDovL3d3dy53My5vcmcvMjAwMC9zdmciIHhtbG5zOnhsaW5rPSJodHRwOi8vd3d3LnczLm9yZy8xOTk5L3hsaW5rIiB2aWV3Qm94PSIwIDAgMTc3LjI1IDQwLjg4Ij48ZGVmcz48c3R5bGU+LmNscy0xe2ZpbGw6dXJsKCNyYWRpYWwtZ3JhZGllbnQpO30uY2xzLTJ7ZmlsbDp1cmwoI2xpbmVhci1ncmFkaWVudCk7fS5jbHMtM3tmaWxsOnVybCgjbGluZWFyLWdyYWRpZW50LTIpO308L3N0eWxlPjxyYWRpYWxHcmFkaWVudCBpZD0icmFkaWFsLWdyYWRpZW50IiBjeD0iOTAuMDkiIGN5PSIyMi42NiIgcj0i ...(+2216 chars)\",\"srcOrientation\":\"Right\"},\"label\":{\"color\":[1,1,0.78,1],\"icon\":{\"size\":[0,0],\"src\":[],\"srcOrientation\":\"Right\"},\"iconPlacement\":\"left\",\"opacity\":1,\"show\":true,\"text\":{\"content\":\"CONFIGURE PLATFORM FOR SENSOR-BASED MOTOR CONTROL\",\"font\":\"Helvetica\",\"fontSize\":2.375646}},\"labelOffset\":[0.025,0],\"verticalAlignment\":\"middle\"},{\"horizontalAlignment\":\"center\",\"image\":{\"position\":[0.04444444444444445,0.005555555555555536,0.9888888888888889,0.9111111111111111],\"size\":[0.9888888888888889,0.9111111111111111],\"src\":\"data:image\\/svg+xml;base64,PHN2ZyB4bWxucz0iaHR0cDovL3d3dy53My5vcmcvMjAwMC9zdmciIHhtbG5zOnhsaW5rPSJodHRwOi8vd3d3LnczLm9yZy8xOTk5L3hsaW5rIiB2aWV3Qm94PSIwIDAgMTc3LjI1IDQwLjg4Ij48ZGVmcz48c3R5bGU+LmNscy0xe2ZpbGw6dXJsKCNyYWRpYWwtZ3JhZGllbnQpO30uY2xzLTJ7ZmlsbDp1cmwoI2xpbmVhci1ncmFkaWVudCk7fS5jbHMtM3tmaWxsOnVybCgjbGluZWFyLWdyYWRpZW50LTIpO308L3N0eWxlPjxyYWRpYWxHcmFkaWVudCBpZD0icmFkaWFsLWdyYWRpZW50IiBjeD0iOTAuMDkiIGN5PSIyMi42NiIgcj0i ...(+2212 chars)\",\"srcOrientation\":\"Right\"},\"label\":{\"color\":[1,1,0.78,1],\"icon\":{\"size\":[0,0],\"src\":[],\"srcOrientation\":\"Right\"},\"iconPlacement\":\"left\",\"opacity\":1,\"show\":true,\"text\":{\"content\":\"CONFIGURE PLATFORM FOR SENSOR-BASED MOTOR CONTROL\",\"font\":\"Helvetica\",\"fontSize\":2.375646}},\"labelOffset\":[0,0],\"verticalAlignment\":\"middle\"},{\"horizontalAlignment\":\"center\",\"image\":{\"position\":[0.04444444444444445,0.005555555555555536,0.9888888888888889,0.9111111111111111],\"size\":[0.9888888888888889,0.9111111111111111],\"src\":\"data:image\\/svg+xml;base64,PHN2ZyB4bWxucz0iaHR0cDovL3d3dy53My5vcmcvMjAwMC9zdmciIHhtbG5zOnhsaW5rPSJodHRwOi8vd3d3LnczLm9yZy8xOTk5L3hsaW5rIiB2aWV3Qm94PSIwIDAgMTc3LjI1IDQwLjg4Ij48ZGVmcz48c3R5bGU+LmNscy0xe2ZpbGw6dXJsKCNyYWRpYWwtZ3JhZGllbnQpO30uY2xzLTJ7ZmlsbDp1cmwoI2xpbmVhci1ncmFkaWVudCk7fS5jbHMtM3tmaWxsOnVybCgjbGluZWFyLWdyYWRpZW50LTIpO308L3N0eWxlPjxyYWRpYWxHcmFkaWVudCBpZD0icmFkaWFsLWdyYWRpZW50IiBjeD0iOTAuMDkiIGN5PSIyMi42NiIgcj0i ...(+2216 chars)\",\"srcOrientation\":\"Right\"},\"label\":{\"color\":[1,1,0.78,1],\"icon\":{\"size\":[0,0],\"src\":[],\"srcOrientation\":\"Right\"},\"iconPlacement\":\"left\",\"opacity\":1,\"show\":true,\"text\":{\"content\":\"CONFIGURE PLATFORM FOR SENSOR-BASED MOTOR CONTROL\",\"font\":\"Helvetica\",\"fontSize\":2.375646}},\"labelOffset\":[0.025,0],\"verticalAlignment\":\"middle\"}]}},{\"name\":\"ForegroundImageComponent\",\"settings\":{\"image\":{\"size\":[0,0],\"src\":\"default\",\"srcOrientation\":\"horizontal\"},\"isForeground\":1,\"position\":[0,0,1,1],\"scaleMode\":\"0\"}}],\"settings\":{\"BindingType\":\"param\",\"aspectRatio\":3.7777777777777777,\"backgroundColor\":[255,255,255,\"1\"],\"backgroundOffset\":0,\"backgroundOpacity\":1,\"fixedAspectRatio\":\"on\",\"foregroundColor\":[252,252,196],\"showBackgroundColor\":false,\"variant\":\"callback\",\"version\":\"R2022b\"},\"type\":\"Button\"}"
  Callback Button4 : CustomCallbackButton  Configuration="{\"components\":[{\"name\":\"BackgroundImageComponent\",\"settings\":{\"image\":{\"size\":[0,0],\"src\":\"default\",\"srcOrientation\":\"horizontal\"},\"position\":[0,0,1,1],\"scaleMode\":\"0\"}},{\"name\":\"ButtonStateComponent\",\"settings\":{\"buttonType\":\"momentary\",\"clickFcn\":\"\\nsave_system;\\n\\nproj = simulinkproject;\\nproj_dir = proj.RootFolder;\\nconfiguration_dd = Simulink.data.dictionary.open([proj_dir,'\\\\data_dictionary\\\\dd_foc_configuration_parameter.sldd']);\\ninterface_dd = Simulink.data.dictionary.open([proj_dir,'\\\\data_dictionary\\\\dd_foc_data_type.sldd']);\\nconfiguration_data_obj = getSection(configuration_dd,'Design Data');\\ninterface_data_obj = getSection(interface_dd,'Design Data');\\n\\n% configure motor control components\\n    %Fast task\\nopen_system([proj_dir,'\\\\referenced_model\\\\ASW_DcycGen\\\\ASW_DcycGen.slx']);\\nmodel_path = 'ASW_DcycGen';\\nset_param([model_path,'\\/DcycGen_FstTask\\/vrs_ModulElecAgCalc'],...\\n    'LabelModeActiveChoice','cstSenlCtrlLbl');\\nset_param([model_path,'\\/DcycGen_FstTask\\/vrs_FstTaskIn'],...\\n    'LabelModeActiveChoice','cstSenlCtrlLbl');\\nset_param([model_path,'\\/DcycGen_FstTask\\/vrs_FstTaskOut'],...\\n    'LabelModeActiveChoice','cstSenlCtrlLbl');\\n\\nsave_system([proj_dir,'\\\\referenced_model\\\\ASW_DcycGen\\\\ASW_DcycGen.slx'],'SaveDirtyReferencedModels',true);\\nclose_system([proj_dir,'\\\\referenced_model\\\\ASW_DcycGen\\\\ASW_DcycGen.slx']);\\n\\nconfigBus_obj = getValue(getEntry(configuration_data_obj,'BUS_DCYCGEN_FST_TASK_IN_SENLVRNT'));\\nbus_entry = getEntry(interface_data_obj,'BUS_DCYCGEN_FST_TASK_IN');\\nnewbus_obj = getValue(bus_entry);\\nnewbus_obj.Elements = configBus_obj.Elements;\\nsetValue(bus_entry,newbus_obj);\\n\\nconfigBus_obj = getValue(getEntry(configuration_data_obj,'BUS_DCYCGEN_FST_TASK_OUT_SENLVRNT'));\\nbus_entry = getEntry(interface_data_obj,'BUS_DCYCGEN_FST_TASK_OUT');\\nnewbus_obj = getValue(bus_entry);\\nnewbus_obj.Elements = configBus_obj.Elements;\\nsetValue(bus_entry,newbus_obj);\\n\\n    %Medium task\\nopen_system([proj_dir,'\\\\referenced_model\\\\ASW_PhVltgGen\\\\ASW_PhVltgGen.slx']);\\nmodel_path = 'ASW_PhVltgGen';\\nset_param([model_path,'\\/PhVltgGen_MedTask\\/vrs_ActElecAgElecSpdCmpt'],...\\n    'LabelModeActiveChoice','cstSenlCtrlLbl');  \\nset_param([model_path,'\\/PhVltgGen_MedTask\\/vrs_ParkTrasf'],...\\n    'LabelModeActiveChoice','cstSenlCtrlLbl'); \\nset_param([model_path,'\\/PhVltgGen_MedTask\\/vrs_CurrCtl'],...\\n    'LabelModeActiveChoice','cstSensCtrlLbl'); \\nset_param([model_path,'\\/PhVltgGen_MedTask\\/vrs_StrtUpElecAgCalc'],...\\n    'LabelModeActiveChoice','cstSenlCtrlLbl'); \\nset_param([model_path,'\\/PhVltgGen_MedTask\\/vrs_MedTaskIn'],...\\n    'LabelModeActiveChoice','cstSenlCtrlLbl');\\nset_param([model_path,'\\/PhVltgGen_MedTask\\/vrs_MedTaskOut'],...\\n    'LabelModeActiveChoice','cstSenlCtrlLbl');\\n\\nsave_system([proj_dir,'\\\\referenced_model\\\\ASW_PhVltgGen\\\\ASW_PhVltgGen.slx'],'SaveDirtyReferencedModels',true);\\nclose_system([proj_dir,'\\\\referenced_model\\\\ASW_PhVltgGen\\\\ASW_PhVltgGen.slx']);\\n\\nconfigBus_obj = getValue(getEntry(configuration_data_obj,'BUS_PHVLTGGEN_MED_TASK_IN_SENLVRNT'));\\nbus_entry = getEntry(interface_data_obj,'BUS_PHVLTGGEN_MED_TASK_IN');\\nnewbus_obj = getValue(bus_entry);\\nnewbus_obj.Elements = configBus_obj.Elements;\\nsetValue(bus_entry,newbus_obj);\\n\\nconfigBus_obj = getValue(getEntry(configuration_data_obj,'BUS_PHVLTGGEN_MED_TASK_OUT_SENLVRNT'));\\nbus_entry = getEntry(interface_data_obj,'BUS_PHVLTGGEN_MED_TASK_OUT');\\nnewbus_obj = getValue(bus_entry);\\nnewbus_obj.Elements = configBus_obj.Elements;\\nsetValue(bus_entry,newbus_obj);\\n\\n    %Slow task\\nopen_system([proj_dir,'\\\\referenced_model\\\\ASW_PhCurrGen\\\\ASW_PhCurrGen.slx']);\\nmodel_path = 'ASW_PhCurrGen';    \\nset_param([model_path,'\\/PhCurrGen_SlwTask\\/vrs_MotoSTM'],...\\n    'LabelModeActiveChoice','cstSenlCtrlLbl');\\nset_param([model_path,'\\/PhCurrGen_SlwTask\\/vrs_StrtUpPrcdChk'],...\\n    'LabelModeActiveChoice','cstSenlCtrlLbl'); \\nset_param([model_path,'\\/PhCurrGen_SlwTask\\/vrs_StrtUpRefTqCalc'],...\\n    'LabelModeActiveChoice','cstSenlCtrlLbl'); \\nset_param([model_path,'\\/PhCurrGen_SlwTask\\/vrs_ElecSpdCtl'],...\\n    'LabelModeActiveChoice','cstSenlCtrlLbl');\\nset_param([model_path,'\\/PhCurrGen_SlwTask\\/vrs_SlwTaskIn'],...\\n    'LabelModeActiveChoice','cstSenlCtrlLbl');  \\nset_param([model_path,'\\/PhCurrGen_SlwTask\\/vrs_SlwTaskOut'],...\\n    'LabelModeActiveChoice','cstSenlCtrlLbl');    \\nsave_system([proj_dir,'\\\\referenced_model\\\\ASW_PhCurrGen\\\\ASW_PhCurrGen.slx'],'SaveDirtyReferencedModels',true);\\nclose_system([proj_dir,'\\\\referenced_model\\\\ASW_PhCurrGen\\\\ASW_PhCurrGen.slx']);\\n\\nconfigBus_obj = getValue(getEntry(configuration_data_obj,'BUS_PHCURRGEN_SLW_TASK_IN_SENLVRNT'));\\nbus_entry = getEntry(interface_data_obj,'BUS_PHCURRGEN_SLW_TASK_IN');\\nnewbus_obj = getValue(bus_entry);\\nnewbus_obj.Elements = configBus_obj.Elements;\\nsetValue(bus_entry,newbus_obj);\\n\\nconfigBus_obj = getValue(getEntry(configuration_data_obj,'BUS_PHCURRGEN_SLW_TASK_OUT_SENLVRNT'));\\nbus_entry = getEntry(interface_data_obj,'BUS_PHCURRGEN_SLW_TASK_OUT');\\nnewbus_obj = getValue(bus_entry);\\nnewbus_obj.Elements = configBus_obj.Elements;\\nsetValue(bus_entry,newbus_obj);\\n\\n% configure assistant components\\nopen_system([proj_dir,'\\\\referenced_model\\\\ASW_AST\\\\ASW_AST.slx']);\\nmodel_path = 'ASW_AST';\\nset_param([model_path,'\\/AST_SlwTask\\/vrs_SensAgCalib'],...\\n    'LabelModeActiveChoice','cstSenlCtrlLbl');\\nset_param([model_path,'\\/AST_SlwTask\\/vrs_RefElecSpdCalc'],...\\n    'LabelModeActiveChoice','cstSenlCtrlLbl');\\nset_param([model_path,'\\/AST_SlwTask\\/vrs_ShOffFlgConf'],...\\n    'LabelModeActiveChoice','cstSenlCtrlLbl');\\nset_param([model_path,'\\/AST_SlwTask\\/vrs_AgEvalModeCalc'],...\\n    'LabelModeActiveChoice','cstSensCtrlLbl');\\nset_param([model_path,'\\/AST_SlwTask\\/vrs_SlwTaskIn'],...\\n    'LabelModeActiveChoice','cstSenlCtrlLbl');\\nset_param([model_path,'\\/AST_SlwTask\\/vrs_SlwTaskOut'],...\\n    'LabelModeActiveChoice','cstSenlCtrlLbl');\\nsave_system([proj_dir,'\\\\referenced_model\\\\ASW_AST\\\\ASW_AST.slx'],'SaveDirtyReferencedModels',true);\\nclose_system([proj_dir,'\\\\referenced_model\\\\ASW_AST\\\\ASW_AST.slx']);\\n\\nconfigBus_obj = getValue(getEntry(configuration_data_obj,'BUS_AST_SLW_TASK_IN_SENLVRNT'));\\nbus_entry = getEntry(interface_data_obj,'BUS_AST_SLW_TASK_IN');\\nnewbus_obj = getValue(bus_entry);\\nnewbus_obj.Elements = configBus_obj.Elements;\\nsetValue(bus_entry,newbus_obj);\\n\\nconfigBus_obj = getValue(getEntry(configuration_data_obj,'BUS_AST_SLW_TASK_OUT_SENLVRNT'));\\nbus_entry = getEntry(interface_data_obj,'BUS_AST_SLW_TASK_OUT');\\nnewbus_obj = getValue(bus_entry);\\nnewbus_obj.Elements = configBus_obj.Elements;\\nsetValue(bus_entry,newbus_obj);\\n\\n\\n% configure OBD components\\nopen_system([proj_dir,'\\\\referenced_model\\\\ASW_OBD\\\\ASW_OBD.slx']);\\nmodel_path = 'ASW_OBD';\\nset_param([model_path,'\\/OBD_SlwTask\\/vrs_MotoStallDia'],...\\n    'LabelModeActiveChoice','cstSenlCtrlLbl');\\nset_param([model_path,'\\/OBD_SlwTask\\/vrs_FaltEnFlgConf'],...\\n    'LabelModeActiveChoice','cstSenlCtrlLbl');\\nset_param([model_path,'\\/OBD_SlwTask\\/vrs_PhiSensFaltDia'],...\\n    'LabelModeActiveChoice','cstSenlCtrlLbl');\\nset_param([model_path,'\\/OBD_SlwTask\\/vrs_SlwTaskIn'],...\\n    'LabelModeActiveChoice','cstSenlCtrlLbl');\\nset_param([model_path,'\\/OBD_SlwTask\\/vrs_SlwTaskOut'],...\\n    'LabelModeActiveChoice','cstSenlCtrlLbl');\\nsave_system([proj_dir,'\\\\referenced_model\\\\ASW_OBD\\\\ASW_OBD.slx'],'SaveDirtyReferencedModels',true);\\nclose_system([proj_dir,'\\\\referenced_model\\\\ASW_OBD\\\\ASW_OBD.slx']);\\n\\nconfigBus_obj = getValue(getEntry(configuration_data_obj,'BUS_OBD_SLW_TASK_IN_SENLVRNT'));\\nbus_entry = getEntry(interface_data_obj,'BUS_OBD_SLW_TASK_IN');\\nnewbus_obj = getValue(bus_entry);\\nnewbus_obj.Elements = configBus_obj.Elements;\\nsetValue(bus_entry,newbus_obj);\\n\\nconfigBus_obj = getValue(getEntry(configuration_data_obj,'BUS_OBD_SLW_TASK_OUT_SENLVRNT'));\\nbus_entry = getEntry(interface_data_obj,'BUS_OBD_SLW_TASK_OUT');\\nnewbus_obj = getValue(bus_entry);\\nnewbus_obj.Elements = configBus_obj.Elements;\\nsetValue(bus_entry,newbus_obj);\\n\\n% configure SigIn componets\\nopen_system([proj_dir,'\\\\referenced_model\\\\ASW_SigIn\\\\ASW_SigIn.slx']);\\nmodel_path = 'ASW_SigIn';\\n    %Medium task\\nset_param([model_path,'\\/SigIn_MedTask\\/vrs_ElecAgCalc'],...\\n    'LabelModeActiveChoice','cstSenlCtrlLbl');\\nset_param([model_path,'\\/SigIn_MedTask\\/vrs_MedTaskIn'],...\\n    'LabelModeActiveChoice','cstSenlCtrlLbl');\\nset_param([model_path,'\\/SigIn_MedTask\\/vrs_MedTaskOut'],...\\n    'LabelModeActiveChoice','cstSenlCtrlLbl');\\n    %Slow task\\nset_param([model_path,'\\/SigIn_SlwTask\\/vrs_SlwTaskOut'],...\\n    'LabelModeActiveChoice','cstSenlCtrlLbl');\\nsave_system([proj_dir,'\\\\referenced_model\\\\ASW_SigIn\\\\ASW_SigIn.slx'],'SaveDirtyReferencedModels',true);\\nclose_system([proj_dir,'\\\\referenced_model\\\\ASW_SigIn\\\\ASW_SigIn.slx']);\\n\\nconfigBus_obj = getValue(getEntry(configuration_data_obj,'BUS_SIGIN_MED_TASK_IN_SENLVRNT'));\\nbus_entry = getEntry(interface_data_obj,'BUS_SIGIN_MED_TASK_IN');\\nnewbus_obj = getValue(bus_entry);\\nnewbus_obj.Elements = configBus_obj.Elements;\\nsetValue(bus_entry,newbus_obj);\\n\\nconfigBus_obj = getValue(getEntry(configuration_data_obj,'BUS_SIGIN_MED_TASK_OUT_SENLVRNT'));\\nbus_entry = getEntry(interface_data_obj,'BUS_SIGIN_MED_TASK_OUT');\\nnewbus_obj = getValue(bus_entry);\\nnewbus_obj.Elements = configBus_obj.Elements;\\nsetValue(bus_entry,newbus_obj);\\n\\nconfigBus_obj = getValue(getEntry(configuration_data_obj,'BUS_SIGIN_SLW_TASK_OUT_SENLVRNT'));\\nbus_entry = getEntry(interface_data_obj,'BUS_SIGIN_SLW_TASK_OUT');\\nnewbus_obj = getValue(bus_entry);\\nnewbus_obj.Elements = configBus_obj.Elements;\\nsetValue(bus_entry,newbus_obj);\\n\\n% configure interfaces of FOC platform\\nopen_system([proj_dir,'\\\\referenced_subsystem\\\\rss_foc_controller_NewPlatform.slx']);\\nmodel_path = 'rss_foc_controller_NewPlatform';\\nset_param([model_path,'\\/vrs_DcycGenFstTaskIn'],'LabelModeActiveChoice','cstSenlCtrlLbl');\\nset_param([model_path,'\\/vrs_DcycGenFstTaskOut'],'LabelModeActiveChoice','cstSenlCtrlLbl');\\nset_param([model_path,'\\/vrs_PhVltgGenMedTaskIn'],'LabelModeActiveChoice','cstSenlCtrlLbl');\\nset_param([model_path,'\\/vrs_PhVltgGenMedTaskOut'],'LabelModeActiveChoice','cstSenlCtrlLbl');\\nset_param([model_path,'\\/vrs_PhCurrGenSlwTaskIn'],'LabelModeActiveChoice','cstSenlCtrlLbl');\\nset_param([model_path,'\\/vrs_PhCurrGenSlwTaskOut'],'LabelModeActiveChoice','cstSenlCtrlLbl');\\nset_param([model_path,'\\/vrs_ASTSlwTaskIn'],'LabelModeActiveChoice','cstSenlCtrlLbl');\\nset_param([model_path,'\\/vrs_ASTSlwTaskOut'],'LabelModeActiveChoice','cstSenlCtrlLbl');\\nset_param([model_path,'\\/vrs_OBDSlwTaskIn'],'LabelModeActiveChoice','cstSenlCtrlLbl');\\nset_param([model_path,'\\/vrs_OBDSlwTaskOut'],'LabelModeActiveChoice','cstSenlCtrlLbl');\\nset_param([model_path,'\\/vrs_SigInMedTaskIn'],'LabelModeActiveChoice','cstSenlCtrlLbl');\\nset_param([model_path,'\\/vrs_SigInMedTaskOut'],'LabelModeActiveChoice','cstSenlCtrlLbl');\\nset_param([model_path,'\\/vrs_SigInSlwTaskOut'],'LabelModeActiveChoice','cstSenlCtrlLbl');\\nsave_system([proj_dir,'\\\\referenced_subsystem\\\\rss_foc_controller_NewPlatform.slx'],'SaveDirtyReferencedModels',true);\\nclose_system([proj_dir,'\\\\referenced_subsystem\\\\rss_foc_controller_NewPlatform.slx']);\",\"image\":{\"size\":[180,45],\"srcOrientation\":\"Right\"},\"onValue\":1,\"position\":[0,0,1,1],\"pressDelay\":\"500\",\"pressFcn\":\"\",\"repeatInterval\":\"0\",\"states\":[{\"horizontalAlignment\":\"center\",\"image\":{\"position\":[0.04444444444444445,0.005555555555555536,0.9888888888888889,0.9111111111111111],\"size\":[0.9888888888888889,0.9111111111111111],\"src\":\"data:image\\/svg+xml;base64,PHN2ZyB4bWxucz0iaHR0cDovL3d3dy53My5vcmcvMjAwMC9zdmciIHhtbG5zOnhsaW5rPSJodHRwOi8vd3d3LnczLm9yZy8xOTk5L3hsaW5rIiB2aWV3Qm94PSIwIDAgMTc3LjI1IDQwLjg4Ij48ZGVmcz48c3R5bGU+LmNscy0xe2ZpbGw6dXJsKCNyYWRpYWwtZ3JhZGllbnQpO30uY2xzLTJ7ZmlsbDp1cmwoI2xpbmVhci1ncmFkaWVudCk7fS5jbHMtM3tmaWxsOnVybCgjbGluZWFyLWdyYWRpZW50LTIpO308L3N0eWxlPjxyYWRpYWxHcmFkaWVudCBpZD0icmFkaWFsLWdyYWRpZW50IiBjeD0iOTAuMDkiIGN5PSIyMi42NiIgcj0i ...(+2212 chars)\",\"srcOrientation\":\"Right\"},\"label\":{\"color\":[1,1,0.78,1],\"icon\":{\"size\":[0,0],\"src\":[],\"srcOrientation\":\"Right\"},\"iconPlacement\":\"left\",\"opacity\":1,\"show\":true,\"text\":{\"content\":\"CONFIGURE PLATFORM FOR SENSOR-LESS MOTOR CONTROL\",\"font\":\"Helvetica\",\"fontSize\":7}},\"labelOffset\":[0,0],\"verticalAlignment\":\"middle\"},{\"horizontalAlignment\":\"center\",\"image\":{\"position\":[0.04444444444444445,0.005555555555555536,0.9888888888888889,0.9111111111111111],\"size\":[0.9888888888888889,0.9111111111111111],\"src\":\"data:image\\/svg+xml;base64,PHN2ZyB4bWxucz0iaHR0cDovL3d3dy53My5vcmcvMjAwMC9zdmciIHhtbG5zOnhsaW5rPSJodHRwOi8vd3d3LnczLm9yZy8xOTk5L3hsaW5rIiB2aWV3Qm94PSIwIDAgMTc3LjI1IDQwLjg4Ij48ZGVmcz48c3R5bGU+LmNscy0xe2ZpbGw6dXJsKCNyYWRpYWwtZ3JhZGllbnQpO30uY2xzLTJ7ZmlsbDp1cmwoI2xpbmVhci1ncmFkaWVudCk7fS5jbHMtM3tmaWxsOnVybCgjbGluZWFyLWdyYWRpZW50LTIpO308L3N0eWxlPjxyYWRpYWxHcmFkaWVudCBpZD0icmFkaWFsLWdyYWRpZW50IiBjeD0iOTAuMDkiIGN5PSIyMi42NiIgcj0i ...(+2216 chars)\",\"srcOrientation\":\"Right\"},\"label\":{\"color\":[1,1,0.78,1],\"icon\":{\"size\":[0,0],\"src\":[],\"srcOrientation\":\"Right\"},\"iconPlacement\":\"left\",\"opacity\":1,\"show\":true,\"text\":{\"content\":\"CONFIGURE PLATFORM FOR SENSOR-LESS MOTOR CONTROL\",\"font\":\"Helvetica\",\"fontSize\":7}},\"labelOffset\":[0.025,0],\"verticalAlignment\":\"middle\"},{\"horizontalAlignment\":\"center\",\"image\":{\"position\":[0.04444444444444445,0.005555555555555536,0.9888888888888889,0.9111111111111111],\"size\":[0.9888888888888889,0.9111111111111111],\"src\":\"data:image\\/svg+xml;base64,PHN2ZyB4bWxucz0iaHR0cDovL3d3dy53My5vcmcvMjAwMC9zdmciIHhtbG5zOnhsaW5rPSJodHRwOi8vd3d3LnczLm9yZy8xOTk5L3hsaW5rIiB2aWV3Qm94PSIwIDAgMTc3LjI1IDQwLjg4Ij48ZGVmcz48c3R5bGU+LmNscy0xe2ZpbGw6dXJsKCNyYWRpYWwtZ3JhZGllbnQpO30uY2xzLTJ7ZmlsbDp1cmwoI2xpbmVhci1ncmFkaWVudCk7fS5jbHMtM3tmaWxsOnVybCgjbGluZWFyLWdyYWRpZW50LTIpO308L3N0eWxlPjxyYWRpYWxHcmFkaWVudCBpZD0icmFkaWFsLWdyYWRpZW50IiBjeD0iOTAuMDkiIGN5PSIyMi42NiIgcj0i ...(+2212 chars)\",\"srcOrientation\":\"Right\"},\"label\":{\"color\":[1,1,0.78,1],\"icon\":{\"size\":[0,0],\"src\":[],\"srcOrientation\":\"Right\"},\"iconPlacement\":\"left\",\"opacity\":1,\"show\":true,\"text\":{\"content\":\"CONFIGURE PLATFORM FOR SENSOR-LESS MOTOR CONTROL\",\"font\":\"Helvetica\",\"fontSize\":7}},\"labelOffset\":[0,0],\"verticalAlignment\":\"middle\"},{\"horizontalAlignment\":\"center\",\"image\":{\"position\":[0.04444444444444445,0.005555555555555536,0.9888888888888889,0.9111111111111111],\"size\":[0.9888888888888889,0.9111111111111111],\"src\":\"data:image\\/svg+xml;base64,PHN2ZyB4bWxucz0iaHR0cDovL3d3dy53My5vcmcvMjAwMC9zdmciIHhtbG5zOnhsaW5rPSJodHRwOi8vd3d3LnczLm9yZy8xOTk5L3hsaW5rIiB2aWV3Qm94PSIwIDAgMTc3LjI1IDQwLjg4Ij48ZGVmcz48c3R5bGU+LmNscy0xe2ZpbGw6dXJsKCNyYWRpYWwtZ3JhZGllbnQpO30uY2xzLTJ7ZmlsbDp1cmwoI2xpbmVhci1ncmFkaWVudCk7fS5jbHMtM3tmaWxsOnVybCgjbGluZWFyLWdyYWRpZW50LTIpO308L3N0eWxlPjxyYWRpYWxHcmFkaWVudCBpZD0icmFkaWFsLWdyYWRpZW50IiBjeD0iOTAuMDkiIGN5PSIyMi42NiIgcj0i ...(+2216 chars)\",\"srcOrientation\":\"Right\"},\"label\":{\"color\":[1,1,0.78,1],\"icon\":{\"size\":[0,0],\"src\":[],\"srcOrientation\":\"Right\"},\"iconPlacement\":\"left\",\"opacity\":1,\"show\":true,\"text\":{\"content\":\"CONFIGURE PLATFORM FOR SENSOR-LESS MOTOR CONTROL\",\"font\":\"Helvetica\",\"fontSize\":7}},\"labelOffset\":[0.025,0],\"verticalAlignment\":\"middle\"}]}},{\"name\":\"ForegroundImageComponent\",\"settings\":{\"image\":{\"size\":[0,0],\"src\":\"default\",\"srcOrientation\":\"horizontal\"},\"isForeground\":1,\"position\":[0,0,1,1],\"scaleMode\":\"0\"}}],\"settings\":{\"BindingType\":\"param\",\"aspectRatio\":3.7777777777777777,\"backgroundColor\":[255,255,255,\"1\"],\"backgroundOffset\":0,\"backgroundOpacity\":1,\"fixedAspectRatio\":\"off\",\"foregroundColor\":[252,252,196],\"showBackgroundColor\":false,\"variant\":\"callback\",\"version\":\"R2022b\"},\"type\":\"Button\"}"
  Callback Button5 : CustomCallbackButton  Configuration="{\"components\":[{\"name\":\"BackgroundImageComponent\",\"settings\":{\"image\":{\"size\":[0,0],\"src\":\"default\",\"srcOrientation\":\"horizontal\"},\"position\":[0,0,1,1],\"scaleMode\":\"0\"}},{\"name\":\"ButtonStateComponent\",\"settings\":{\"buttonType\":\"momentary\",\"clickFcn\":\"\\nsave_system;\\n\\nproj = simulinkproject;\\nproj_dir = proj.RootFolder;\\nconfiguration_dd = Simulink.data.dictionary.open([proj_dir,'\\\\data_dictionary\\\\dd_foc_configuration_parameter.sldd']);\\ninterface_dd = Simulink.data.dictionary.open([proj_dir,'\\\\data_dictionary\\\\dd_foc_data_type.sldd']);\\nconfiguration_data_obj = getSection(configuration_dd,'Design Data');\\ninterface_data_obj = getSection(interface_dd,'Design Data');\\n\\n% configure motor control components\\n    %Fast task\\nopen_system([proj_dir,'\\\\referenced_model\\\\ASW_DcycGen\\\\ASW_DcycGen.slx']);\\nmodel_path = 'ASW_DcycGen';\\nset_param([model_path,'\\/DcycGen_FstTask\\/vrs_ModulElecAgCalc'],...\\n    'LabelModeActiveChoice','cstSensCtrlLbl');\\nset_param([model_path,'\\/DcycGen_FstTask\\/vrs_FstTaskIn'],...\\n    'LabelModeActiveChoice','cstSensCtrlLbl');\\nset_param([model_path,'\\/DcycGen_FstTask\\/vrs_FstTaskOut'],...\\n    'LabelModeActiveChoice','cstSensCtrlLbl');\\n\\nsave_system([proj_dir,'\\\\referenced_model\\\\ASW_DcycGen\\\\ASW_DcycGen.slx'],'SaveDirtyReferencedModels',true);\\nclose_system([proj_dir,'\\\\referenced_model\\\\ASW_DcycGen\\\\ASW_DcycGen.slx']);\\n\\nconfigBus_obj = getValue(getEntry(configuration_data_obj,'BUS_DCYCGEN_FST_TASK_IN_SENSVRNT'));\\nbus_entry = getEntry(interface_data_obj,'BUS_DCYCGEN_FST_TASK_IN');\\nnewbus_obj = getValue(bus_entry);\\nnewbus_obj.Elements = configBus_obj.Elements;\\nsetValue(bus_entry,newbus_obj);\\n\\nconfigBus_obj = getValue(getEntry(configuration_data_obj,'BUS_DCYCGEN_FST_TASK_OUT_SENSVRNT'));\\nbus_entry = getEntry(interface_data_obj,'BUS_DCYCGEN_FST_TASK_OUT');\\nnewbus_obj = getValue(bus_entry);\\nnewbus_obj.Elements = configBus_obj.Elements;\\nsetValue(bus_entry,newbus_obj);\\n\\n    %Medium task\\nopen_system([proj_dir,'\\\\referenced_model\\\\ASW_PhVltgGen\\\\ASW_PhVltgGen.slx']);\\nmodel_path = 'ASW_PhVltgGen';\\nset_param([model_path,'\\/PhVltgGen_MedTask\\/vrs_ActElecAgElecSpdCmpt'],...\\n    'LabelModeActiveChoice','cstHybrCtrlLbl');  \\nset_param([model_path,'\\/PhVltgGen_MedTask\\/vrs_ParkTrasf'],...\\n    'LabelModeActiveChoice','cstHybrCtrlLbl'); \\nset_param([model_path,'\\/PhVltgGen_MedTask\\/vrs_CurrCtl'],...\\n    'LabelModeActiveChoice','cstSensCtrlLbl'); \\nset_param([model_path,'\\/PhVltgGen_MedTask\\/vrs_StrtUpElecAgCalc'],...\\n    'LabelModeActiveChoice','cstSenlCtrlLbl'); \\nset_param([model_path,'\\/PhVltgGen_MedTask\\/vrs_MedTaskIn'],...\\n    'LabelModeActiveChoice','cstHybrCtrlLbl');\\nset_param([model_path,'\\/PhVltgGen_MedTask\\/vrs_MedTaskOut'],...\\n    'LabelModeActiveChoice','cstHybrCtrlLbl');\\n\\nsave_system([proj_dir,'\\\\referenced_model\\\\ASW_PhVltgGen\\\\ASW_PhVltgGen.slx'],'SaveDirtyReferencedModels',true);\\nclose_system([proj_dir,'\\\\referenced_model\\\\ASW_PhVltgGen\\\\ASW_PhVltgGen.slx']);\\n\\nconfigBus_obj = getValue(getEntry(configuration_data_obj,'BUS_PHVLTGGEN_MED_TASK_IN_HYBRVRNT'));\\nbus_entry = getEntry(interface_data_obj,'BUS_PHVLTGGEN_MED_TASK_IN');\\nnewbus_obj = getValue(bus_entry);\\nnewbus_obj.Elements = configBus_obj.Elements;\\nsetValue(bus_entry,newbus_obj);\\n\\nconfigBus_obj = getValue(getEntry(configuration_data_obj,'BUS_PHVLTGGEN_MED_TASK_OUT_HYBRVRNT'));\\nbus_entry = getEntry(interface_data_obj,'BUS_PHVLTGGEN_MED_TASK_OUT');\\nnewbus_obj = getValue(bus_entry);\\nnewbus_obj.Elements = configBus_obj.Elements;\\nsetValue(bus_entry,newbus_obj);\\n\\n    %Slow task\\nopen_system([proj_dir,'\\\\referenced_model\\\\ASW_PhCurrGen\\\\ASW_PhCurrGen.slx']);\\nmodel_path = 'ASW_PhCurrGen';    \\nset_param([model_path,'\\/PhCurrGen_SlwTask\\/vrs_MotoSTM'],...\\n    'LabelModeActiveChoice','cstHybrCtrlLbl');\\nset_param([model_path,'\\/PhCurrGen_SlwTask\\/vrs_StrtUpPrcdChk'],...\\n    'LabelModeActiveChoice','cstSenlCtrlLbl'); \\nset_param([model_path,'\\/PhCurrGen_SlwTask\\/vrs_StrtUpRefTqCalc'],...\\n    'LabelModeActiveChoice','cstSenlCtrlLbl'); \\nset_param([model_path,'\\/PhCurrGen_SlwTask\\/vrs_ElecSpdCtl'],...\\n    'LabelModeActiveChoice','cstHybrCtrlLbl');\\nset_param([model_path,'\\/PhCurrGen_SlwTask\\/vrs_SlwTaskIn'],...\\n    'LabelModeActiveChoice','cstHybrCtrlLbl');  \\nset_param([model_path,'\\/PhCurrGen_SlwTask\\/vrs_SlwTaskOut'],...\\n    'LabelModeActiveChoice','cstSenlCtrlLbl');    \\nsave_system([proj_dir,'\\\\referenced_model\\\\ASW_PhCurrGen\\\\ASW_PhCurrGen.slx'],'SaveDirtyReferencedModels',true);\\nclose_system([proj_dir,'\\\\referenced_model\\\\ASW_PhCurrGen\\\\ASW_PhCurrGen.slx']);\\n\\nconfigBus_obj = getValue(getEntry(configuration_data_obj,'BUS_PHCURRGEN_SLW_TASK_IN_HYBRVRNT'));\\nbus_entry = getEntry(interface_data_obj,'BUS_PHCURRGEN_SLW_TASK_IN');\\nnewbus_obj = getValue(bus_entry);\\nnewbus_obj.Elements = configBus_obj.Elements;\\nsetValue(bus_entry,newbus_obj);\\n\\nconfigBus_obj = getValue(getEntry(configuration_data_obj,'BUS_PHCURRGEN_SLW_TASK_OUT_SENLVRNT'));\\nbus_entry = getEntry(interface_data_obj,'BUS_PHCURRGEN_SLW_TASK_OUT');\\nnewbus_obj = getValue(bus_entry);\\nnewbus_obj.Elements = configBus_obj.Elements;\\nsetValue(bus_entry,newbus_obj);\\n\\n% configure assistant components\\nopen_system([proj_dir,'\\\\referenced_model\\\\ASW_AST\\\\ASW_AST.slx']);\\nmodel_path = 'ASW_AST';\\nset_param([model_path,'\\/AST_SlwTask\\/vrs_SensAgCalib'],...\\n    'LabelModeActiveChoice','cstSensCtrlLbl');\\nset_param([model_path,'\\/AST_SlwTask\\/vrs_RefElecSpdCalc'],...\\n    'LabelModeActiveChoice','cstHybrCtrlLbl');\\nset_param([model_path,'\\/AST_SlwTask\\/vrs_ShOffFlgConf'],...\\n    'LabelModeActiveChoice','cstSensCtrlLbl');\\nset_param([model_path,'\\/AST_SlwTask\\/vrs_AgEvalModeCalc'],...\\n    'LabelModeActiveChoice','cstHybrCtrlLbl');\\nset_param([model_path,'\\/AST_SlwTask\\/vrs_SlwTaskIn'],...\\n    'LabelModeActiveChoice','cstHybrCtrlLbl');\\nset_param([model_path,'\\/AST_SlwTask\\/vrs_SlwTaskOut'],...\\n    'LabelModeActiveChoice','cstHybrCtrlLbl');\\nsave_system([proj_dir,'\\\\referenced_model\\\\ASW_AST\\\\ASW_AST.slx'],'SaveDirtyReferencedModels',true);\\nclose_system([proj_dir,'\\\\referenced_model\\\\ASW_AST\\\\ASW_AST.slx']);\\n\\nconfigBus_obj = getValue(getEntry(configuration_data_obj,'BUS_AST_SLW_TASK_IN_HYBRVRNT'));\\nbus_entry = getEntry(interface_data_obj,'BUS_AST_SLW_TASK_IN');\\nnewbus_obj = getValue(bus_entry);\\nnewbus_obj.Elements = configBus_obj.Elements;\\nsetValue(bus_entry,newbus_obj);\\n\\nconfigBus_obj = getValue(getEntry(configuration_data_obj,'BUS_AST_SLW_TASK_OUT_HYBRVRNT'));\\nbus_entry = getEntry(interface_data_obj,'BUS_AST_SLW_TASK_OUT');\\nnewbus_obj = getValue(bus_entry);\\nnewbus_obj.Elements = configBus_obj.Elements;\\nsetValue(bus_entry,newbus_obj);\\n\\n\\n% configure OBD components\\nopen_system([proj_dir,'\\\\referenced_model\\\\ASW_OBD\\\\ASW_OBD.slx']);\\nmodel_path = 'ASW_OBD';\\nset_param([model_path,'\\/OBD_SlwTask\\/vrs_MotoStallDia'],...\\n    'LabelModeActiveChoice','cstHybrCtrlLbl');\\nset_param([model_path,'\\/OBD_SlwTask\\/vrs_FaltEnFlgConf'],...\\n    'LabelModeActiveChoice','cstSenlCtrlLbl');\\nset_param([model_path,'\\/OBD_SlwTask\\/vrs_PhiSensFaltDia'],...\\n    'LabelModeActiveChoice','cstHybrCtrlLbl');\\nset_param([model_path,'\\/OBD_SlwTask\\/vrs_SlwTaskIn'],...\\n    'LabelModeActiveChoice','cstHybrCtrlLbl');\\nset_param([model_path,'\\/OBD_SlwTask\\/vrs_SlwTaskOut'],...\\n    'LabelModeActiveChoice','cstHybrCtrlLbl');\\nsave_system([proj_dir,'\\\\referenced_model\\\\ASW_OBD\\\\ASW_OBD.slx'],'SaveDirtyReferencedModels',true);\\nclose_system([proj_dir,'\\\\referenced_model\\\\ASW_OBD\\\\ASW_OBD.slx']);\\n\\nconfigBus_obj = getValue(getEntry(configuration_data_obj,'BUS_OBD_SLW_TASK_IN_HYBRVRNT'));\\nbus_entry = getEntry(interface_data_obj,'BUS_OBD_SLW_TASK_IN');\\nnewbus_obj = getValue(bus_entry);\\nnewbus_obj.Elements = configBus_obj.Elements;\\nsetValue(bus_entry,newbus_obj);\\n\\nconfigBus_obj = getValue(getEntry(configuration_data_obj,'BUS_OBD_SLW_TASK_OUT_HYBRVRNT'));\\nbus_entry = getEntry(interface_data_obj,'BUS_OBD_SLW_TASK_OUT');\\nnewbus_obj = getValue(bus_entry);\\nnewbus_obj.Elements = configBus_obj.Elements;\\nsetValue(bus_entry,newbus_obj);\\n\\n% configure SigIn componets\\nopen_system([proj_dir,'\\\\referenced_model\\\\ASW_SigIn\\\\ASW_SigIn.slx']);\\nmodel_path = 'ASW_SigIn';\\n    %Medium task\\nset_param([model_path,'\\/SigIn_MedTask\\/vrs_ElecAgCalc'],...\\n    'LabelModeActiveChoice','cstSensCtrlLbl');\\nset_param([model_path,'\\/SigIn_MedTask\\/vrs_MedTaskIn'],...\\n    'LabelModeActiveChoice','cstSensCtrlLbl');\\nset_param([model_path,'\\/SigIn_MedTask\\/vrs_MedTaskOut'],...\\n    'LabelModeActiveChoice','cstSensCtrlLbl');\\n    %Slow task\\nset_param([model_path,'\\/SigIn_SlwTask\\/vrs_SlwTaskOut'],...\\n    'LabelModeActiveChoice','cstSenlCtrlLbl');\\nsave_system([proj_dir,'\\\\referenced_model\\\\ASW_SigIn\\\\ASW_SigIn.slx'],'SaveDirtyReferencedModels',true);\\nclose_system([proj_dir,'\\\\referenced_model\\\\ASW_SigIn\\\\ASW_SigIn.slx']);\\n\\nconfigBus_obj = getValue(getEntry(configuration_data_obj,'BUS_SIGIN_MED_TASK_IN_SENSVRNT'));\\nbus_entry = getEntry(interface_data_obj,'BUS_SIGIN_MED_TASK_IN');\\nnewbus_obj = getValue(bus_entry);\\nnewbus_obj.Elements = configBus_obj.Elements;\\nsetValue(bus_entry,newbus_obj);\\n\\nconfigBus_obj = getValue(getEntry(configuration_data_obj,'BUS_SIGIN_MED_TASK_OUT_SENSVRNT'));\\nbus_entry = getEntry(interface_data_obj,'BUS_SIGIN_MED_TASK_OUT');\\nnewbus_obj = getValue(bus_entry);\\nnewbus_obj.Elements = configBus_obj.Elements;\\nsetValue(bus_entry,newbus_obj);\\n\\nconfigBus_obj = getValue(getEntry(configuration_data_obj,'BUS_SIGIN_SLW_TASK_OUT_SENLVRNT'));\\nbus_entry = getEntry(interface_data_obj,'BUS_SIGIN_SLW_TASK_OUT');\\nnewbus_obj = getValue(bus_entry);\\nnewbus_obj.Elements = configBus_obj.Elements;\\nsetValue(bus_entry,newbus_obj);\\n\\n% configure interfaces of FOC platform\\nopen_system([proj_dir,'\\\\referenced_subsystem\\\\rss_foc_controller_NewPlatform.slx']);\\nmodel_path = 'rss_foc_controller_NewPlatform';\\nset_param([model_path,'\\/vrs_DcycGenFstTaskIn'],'LabelModeActiveChoice','cstSensCtrlLbl');\\nset_param([model_path,'\\/vrs_DcycGenFstTaskOut'],'LabelModeActiveChoice','cstSensCtrlLbl');\\nset_param([model_path,'\\/vrs_PhVltgGenMedTaskIn'],'LabelModeActiveChoice','cstHybrCtrlLbl');\\nset_param([model_path,'\\/vrs_PhVltgGenMedTaskOut'],'LabelModeActiveChoice','cstHybrCtrlLbl');\\nset_param([model_path,'\\/vrs_PhCurrGenSlwTaskIn'],'LabelModeActiveChoice','cstHybrCtrlLbl');\\nset_param([model_path,'\\/vrs_PhCurrGenSlwTaskOut'],'LabelModeActiveChoice','cstSenlCtrlLbl');\\nset_param([model_path,'\\/vrs_ASTSlwTaskIn'],'LabelModeActiveChoice','cstHybrCtrlLbl');\\nset_param([model_path,'\\/vrs_ASTSlwTaskOut'],'LabelModeActiveChoice','cstHybrCtrlLbl');\\nset_param([model_path,'\\/vrs_OBDSlwTaskIn'],'LabelModeActiveChoice','cstHybrCtrlLbl');\\nset_param([model_path,'\\/vrs_OBDSlwTaskOut'],'LabelModeActiveChoice','cstHybrCtrlLbl');\\nset_param([model_path,'\\/vrs_SigInMedTaskIn'],'LabelModeActiveChoice','cstSensCtrlLbl');\\nset_param([model_path,'\\/vrs_SigInMedTaskOut'],'LabelModeActiveChoice','cstSensCtrlLbl');\\nset_param([model_path,'\\/vrs_SigInSlwTaskOut'],'LabelModeActiveChoice','cstSenlCtrlLbl');\\nsave_system([proj_dir,'\\\\referenced_subsystem\\\\rss_foc_controller_NewPlatform.slx'],'SaveDirtyReferencedModels',true);\\nclose_system([proj_dir,'\\\\referenced_subsystem\\\\rss_foc_controller_NewPlatform.slx']);\",\"image\":{\"size\":[180,45],\"srcOrientation\":\"Right\"},\"onValue\":1,\"position\":[0,0,1,1],\"pressDelay\":\"500\",\"pressFcn\":\"\",\"repeatInterval\":\"0\",\"states\":[{\"horizontalAlignment\":\"center\",\"image\":{\"position\":[0.04444444444444445,0.005555555555555536,0.9888888888888889,0.9111111111111111],\"size\":[0.9888888888888889,0.9111111111111111],\"src\":\"data:image\\/svg+xml;base64,PHN2ZyB4bWxucz0iaHR0cDovL3d3dy53My5vcmcvMjAwMC9zdmciIHhtbG5zOnhsaW5rPSJodHRwOi8vd3d3LnczLm9yZy8xOTk5L3hsaW5rIiB2aWV3Qm94PSIwIDAgMTc3LjI1IDQwLjg4Ij48ZGVmcz48c3R5bGU+LmNscy0xe2ZpbGw6dXJsKCNyYWRpYWwtZ3JhZGllbnQpO30uY2xzLTJ7ZmlsbDp1cmwoI2xpbmVhci1ncmFkaWVudCk7fS5jbHMtM3tmaWxsOnVybCgjbGluZWFyLWdyYWRpZW50LTIpO308L3N0eWxlPjxyYWRpYWxHcmFkaWVudCBpZD0icmFkaWFsLWdyYWRpZW50IiBjeD0iOTAuMDkiIGN5PSIyMi42NiIgcj0i ...(+2212 chars)\",\"srcOrientation\":\"Right\"},\"label\":{\"color\":[1,1,0.78,1],\"icon\":{\"size\":[0,0],\"src\":[],\"srcOrientation\":\"Right\"},\"iconPlacement\":\"left\",\"opacity\":1,\"show\":true,\"text\":{\"content\":\"CONFIGURE PLATFORM FOR HYBRID MOTOR CONTROL\",\"font\":\"Helvetica\",\"fontSize\":7}},\"labelOffset\":[0,0],\"verticalAlignment\":\"middle\"},{\"horizontalAlignment\":\"center\",\"image\":{\"position\":[0.04444444444444445,0.005555555555555536,0.9888888888888889,0.9111111111111111],\"size\":[0.9888888888888889,0.9111111111111111],\"src\":\"data:image\\/svg+xml;base64,PHN2ZyB4bWxucz0iaHR0cDovL3d3dy53My5vcmcvMjAwMC9zdmciIHhtbG5zOnhsaW5rPSJodHRwOi8vd3d3LnczLm9yZy8xOTk5L3hsaW5rIiB2aWV3Qm94PSIwIDAgMTc3LjI1IDQwLjg4Ij48ZGVmcz48c3R5bGU+LmNscy0xe2ZpbGw6dXJsKCNyYWRpYWwtZ3JhZGllbnQpO30uY2xzLTJ7ZmlsbDp1cmwoI2xpbmVhci1ncmFkaWVudCk7fS5jbHMtM3tmaWxsOnVybCgjbGluZWFyLWdyYWRpZW50LTIpO308L3N0eWxlPjxyYWRpYWxHcmFkaWVudCBpZD0icmFkaWFsLWdyYWRpZW50IiBjeD0iOTAuMDkiIGN5PSIyMi42NiIgcj0i ...(+2216 chars)\",\"srcOrientation\":\"Right\"},\"label\":{\"color\":[1,1,0.78,1],\"icon\":{\"size\":[0,0],\"src\":[],\"srcOrientation\":\"Right\"},\"iconPlacement\":\"left\",\"opacity\":1,\"show\":true,\"text\":{\"content\":\"CONFIGURE PLATFORM FOR HYBRID MOTOR CONTROL\",\"font\":\"Helvetica\",\"fontSize\":7}},\"labelOffset\":[0.025,0],\"verticalAlignment\":\"middle\"},{\"horizontalAlignment\":\"center\",\"image\":{\"position\":[0.04444444444444445,0.005555555555555536,0.9888888888888889,0.9111111111111111],\"size\":[0.9888888888888889,0.9111111111111111],\"src\":\"data:image\\/svg+xml;base64,PHN2ZyB4bWxucz0iaHR0cDovL3d3dy53My5vcmcvMjAwMC9zdmciIHhtbG5zOnhsaW5rPSJodHRwOi8vd3d3LnczLm9yZy8xOTk5L3hsaW5rIiB2aWV3Qm94PSIwIDAgMTc3LjI1IDQwLjg4Ij48ZGVmcz48c3R5bGU+LmNscy0xe2ZpbGw6dXJsKCNyYWRpYWwtZ3JhZGllbnQpO30uY2xzLTJ7ZmlsbDp1cmwoI2xpbmVhci1ncmFkaWVudCk7fS5jbHMtM3tmaWxsOnVybCgjbGluZWFyLWdyYWRpZW50LTIpO308L3N0eWxlPjxyYWRpYWxHcmFkaWVudCBpZD0icmFkaWFsLWdyYWRpZW50IiBjeD0iOTAuMDkiIGN5PSIyMi42NiIgcj0i ...(+2212 chars)\",\"srcOrientation\":\"Right\"},\"label\":{\"color\":[1,1,0.78,1],\"icon\":{\"size\":[0,0],\"src\":[],\"srcOrientation\":\"Right\"},\"iconPlacement\":\"left\",\"opacity\":1,\"show\":true,\"text\":{\"content\":\"CONFIGURE PLATFORM FOR HYBRID MOTOR CONTROL\",\"font\":\"Helvetica\",\"fontSize\":7}},\"labelOffset\":[0,0],\"verticalAlignment\":\"middle\"},{\"horizontalAlignment\":\"center\",\"image\":{\"position\":[0.04444444444444445,0.005555555555555536,0.9888888888888889,0.9111111111111111],\"size\":[0.9888888888888889,0.9111111111111111],\"src\":\"data:image\\/svg+xml;base64,PHN2ZyB4bWxucz0iaHR0cDovL3d3dy53My5vcmcvMjAwMC9zdmciIHhtbG5zOnhsaW5rPSJodHRwOi8vd3d3LnczLm9yZy8xOTk5L3hsaW5rIiB2aWV3Qm94PSIwIDAgMTc3LjI1IDQwLjg4Ij48ZGVmcz48c3R5bGU+LmNscy0xe2ZpbGw6dXJsKCNyYWRpYWwtZ3JhZGllbnQpO30uY2xzLTJ7ZmlsbDp1cmwoI2xpbmVhci1ncmFkaWVudCk7fS5jbHMtM3tmaWxsOnVybCgjbGluZWFyLWdyYWRpZW50LTIpO308L3N0eWxlPjxyYWRpYWxHcmFkaWVudCBpZD0icmFkaWFsLWdyYWRpZW50IiBjeD0iOTAuMDkiIGN5PSIyMi42NiIgcj0i ...(+2216 chars)\",\"srcOrientation\":\"Right\"},\"label\":{\"color\":[1,1,0.78,1],\"icon\":{\"size\":[0,0],\"src\":[],\"srcOrientation\":\"Right\"},\"iconPlacement\":\"left\",\"opacity\":1,\"show\":true,\"text\":{\"content\":\"CONFIGURE PLATFORM FOR HYBRID MOTOR CONTROL\",\"font\":\"Helvetica\",\"fontSize\":7}},\"labelOffset\":[0.025,0],\"verticalAlignment\":\"middle\"}]}},{\"name\":\"ForegroundImageComponent\",\"settings\":{\"image\":{\"size\":[0,0],\"src\":\"default\",\"srcOrientation\":\"horizontal\"},\"isForeground\":1,\"position\":[0,0,1,1],\"scaleMode\":\"0\"}}],\"settings\":{\"BindingType\":\"param\",\"aspectRatio\":3.7777777777777777,\"backgroundColor\":[255,255,255,\"1\"],\"backgroundOffset\":0,\"backgroundOpacity\":1,\"fixedAspectRatio\":\"off\",\"foregroundColor\":[252,252,196],\"showBackgroundColor\":false,\"variant\":\"callback\",\"version\":\"R2022b\"},\"type\":\"Button\"}"
  Constant{,3,6..7,10..11,20,25,30,32,34,36,38,41,43,48} (16 alike) : Constant  Value=false  OutDataTypeStr=boolean
  Constant1 : Constant  Value=1024  OutDataTypeStr=uint16
  Constant{12..14,45} (4 alike) : Constant  Value=25  OutDataTypeStr=double
  Constant15 : Constant  Value=10  OutDataTypeStr=uint8
  Constant17 : Constant  Value=0  OutDataTypeStr=uint32
  Constant{18,24,26..27} (4 alike) : Constant  Value=0  OutDataTypeStr=Inherit: Inherit via back propagation
  Constant{4,8..9,19,21,29,31,33,35,37,39..40,42,44,47} (15 alike) : Constant  Value=true  OutDataTypeStr=boolean
  Constant2 : Constant  Value=0  OutDataTypeStr=uint8
  Constant22 : Constant  Value=10  OutDataTypeStr=uint8
  Constant23 : Constant  Value=0  OutDataTypeStr=dt_Temp_u8p0bn40
  Constant28 : Constant  Value=0  OutDataTypeStr=uint32
  Constant46 : Constant  Value=0  OutDataTypeStr=double
  Constant5 : Constant  OutDataTypeStr=double
  CtlBrdVoltage[V] : Constant  Value=14
  Data Type Conversion : DataTypeConversion  OutDataTypeStr=int16  SaturateOnIntegerOverflow=off  RndMeth=Floor
  Data Type Conversion{1,3,5..6,10..13} (8 alike) : DataTypeConversion  OutDataTypeStr=uint16  SaturateOnIntegerOverflow=off  RndMeth=Floor
  Data Type Conversion2 : DataTypeConversion  OutDataTypeStr=uint8  SaturateOnIntegerOverflow=off  RndMeth=Floor
  Data Type Conversion4 : DataTypeConversion  OutDataTypeStr=dt_Temp_u8p0bn40  SaturateOnIntegerOverflow=off  RndMeth=Floor
  Data Type Conversion7 : DataTypeConversion  OutDataTypeStr=dt_RadAng_u16r15b0  SaturateOnIntegerOverflow=off  RndMeth=Floor
  Data Type Conversion9 : DataTypeConversion  OutDataTypeStr=uint8  SaturateOnIntegerOverflow=off  RndMeth=Floor
  Edit : EditField  LabelPosition=Hide  ShowInitialText=on  Alignment=Center
  Edit1 : EditField  LabelPosition=Hide  ShowInitialText=on  Alignment=Center
  From24 : From  Commented=on  GotoTag=iActXYZPhsCurr
  From25 : From  Commented=on  GotoTag=arActMechAng
  From26 : From  Commented=on  GotoTag=tcMagTemp
  GDVoltage : Subsystem
  GDVoltage1 : Subsystem
  GDVoltage[V]1 : Constant  Value=14
  Gain : Gain  Gain=30/pi
  Gain1 : Gain  Gain=30/pi
  Gain2 : Gain  Gain=65535/(2*pi)  OutDataTypeStr=uint16
  Gain3 : Gain  Gain=5
  LoadTorque[Nm] : Constant  Value=0.6080854309687262
  MCUOpMode : Constant
  MCUOpModeHMI : EditField  LabelPosition=Hide  ShowInitialText=on  Alignment=Center
  MagnetTemperatureHMI[°C] : EditField  LabelPosition=Hide  ShowInitialText=on  Alignment=Center
  MagnetTemperature[°C] : Constant  Value=20
  Manual Switch{1..3,5,8..15,17} (13 alike) : ManualSwitch
  Manual Switch6 : ManualSwitch  CurrentSetting=0
  Manual Switch7 : ManualSwitch  CurrentSetting=0
  Mux : Mux  Inputs=2
  Mux1 : Mux  Inputs=2
  Observer : ObserverReference  Commented=on  ObserverModelName=obs_foc_controller
  Rate Transition9 : RateTransition  Commented=through  Deterministic=off
  Scope : Scope  NumInputPorts=4
  Slider : SliderBlock  LabelPosition=Hide  ScaleMax=0.8  TickInterval=0.1
  SupplyVoltage : Subsystem
  SupplyVoltageHMI[V] : EditField  LabelPosition=Hide  ShowInitialText=on  Alignment=Center
  SupplyVoltage[V] : Constant  Value=14
  TargetSpeedHMI[rpm] : EditField  LabelPosition=Hide  ShowInitialText=on  Alignment=Center
  TargetSpeed[rpm] : Constant  Value=4500
  Temperature : Subsystem
  Terminator{,1..5} (6 alike) : Terminator
  WindingTemperatureHMI[°C] : EditField  LabelPosition=Hide  ShowInitialText=on  Alignment=Center
  WindingTemperature[°C] : Constant  Value=20
  XYZPhaseCurrent : Subsystem
  genRlctTrqPerc : Display  Commented=on
  iActPhsCurr : Display
  iEstSplyCurr : Display
  iRealDirCurr : Display  Commented=on
  iRealPhsCurr : Display  Commented=on
  iRealQdrtCurr : Display  Commented=on
  nRefMechSpd : Display
  rss_FocController : Subsystem  TreatAsAtomicUnit=on  ReferencedSubsystem=rss_foc_controller_NewPlatform
  rss_InverterModel : Subsystem  TreatAsAtomicUnit=on  ReferencedSubsystem=rss_inverter_model
  rss_LoadModel : Subsystem  ReferencedSubsystem=rss_load_model
  rss_MotorModel : Subsystem  InitFcn=|  ReferencedSubsystem=rss_motor_model
      | Simulink.suppressDiagnostic([gcb,'/vss_MotorModel/vss_ComplexModelVersion1/Data Type Conversion2'],...
      |  'SimulinkFixedPoint:util:Overflowoccurred');
  sss_CommunicationCommand : Subsystem
  sss_CommunicationError : Subsystem
  sss_SimulationResult : Subsystem  Commented=on  ClipboardFcn=|
      | Simulink.suppressDiagnostic([gcb,'/sss_ParkTransform/Data Type Conversion2'],...
      |  'SimulinkFixedPoint:util:Overflowoccurred');
  tqElctDirTrq : Display  Commented=on
  tqElctRlctTrq : Display  Commented=on
  tqElctTotTrq : Display  Commented=on
  tqLoadTrq : Display
  tqMotTrq : Display
  wActMechSpd : Display
  wElctMechSpd : Display
  wires:
  WindingTemperature[°C]/1 -> [tcWindTemp]
  MagnetTemperature[°C]/1 -> [tcMagTemp]
  TargetSpeed[rpm]/1 -> [nRefMechSpd]
  rss_InverterModel/1 -> [vtXYZPhsVolt]
  rss_FocController/1 -> [genXYZDutyCycl]
  rss_MotorModel/1 -> [iActXYZPhsCurr]
  rss_MotorModel/2 -> [arActMechAng]
  rss_MotorModel/3 -> [wActMechSpd]
  rss_MotorModel/4 -> [tqMotTrq]
  SupplyVoltage[V]/1 -> [vtSplyVolt]
  [nRefMechSpd] -> Mux/1  "nRefMechSpd[rpm]"
  [genXYZDutyCycl] -> Rate Transition9/1  "genXYZDutyCycl[V]"
  Mux/1 -> Scope/3
  Gain/1 -> Mux/2  "nActMechSpd[rpm]"
  [iActXYZPhsCurr] -> Scope/1  "iActXYZPhsCurr[A]"
  [wActMechSpd] -> Gain/1
  [wActMechSpd] -> Gain1/1
  [nRefMechSpd] -> nRefMechSpd/1
  Gain1/1 -> wActMechSpd/1
  [tqLoadTrq] -> tqLoadTrq/1
  [tqMotTrq] -> tqMotTrq/1
  [tqMotTrq] -> Mux1/1  "tqMotTrq[Nm]"
  Mux1/1 -> Scope/4
  [tqLoadTrq] -> Mux1/2  "tqLoadTrq[Nm]"
  sss_SimulationResult/1(iRealPhsCurr) -> iRealPhsCurr/1
  From25/1 -> sss_SimulationResult/1(arMechAng)
  From24/1 -> sss_SimulationResult/2(iActXYZPhsCurr)
  From26/1 -> sss_SimulationResult/3(tcActMagTemp)
  sss_SimulationResult/2(iRealDirCurr) -> iRealDirCurr/1
  sss_SimulationResult/3(iRealQdrtCurr) -> iRealQdrtCurr/1
  sss_SimulationResult/4(tqElctRlctTrq) -> tqElctRlctTrq/1
  sss_SimulationResult/5(tqElctDirTrq) -> tqElctDirTrq/1
  sss_SimulationResult/6(tqElctTotTrq) -> tqElctTotTrq/1
  sss_SimulationResult/7(genRlctTrqPerc) -> genRlctTrqPerc/1
  rss_FocController/6 -> [iEstSplyCurr]
  [iEstSplyCurr] -> iEstSplyCurr/1
  [iActXYZPhsCurr] -> XYZPhaseCurrent/1(iActXYZCurr)
  [vtSplyVolt] -> SupplyVoltage/1(vtSplyVolt)
  Data Type Conversion5/1 -> rss_FocController/7
  Data Type Conversion6/1 -> rss_FocController/3
  [arActMechAng] -> Gain2/1
  Gain2/1 -> Data Type Conversion6/1
  [wActMechSpd] -> Gain3/1
  Gain3/1 -> wElctMechSpd/1
  [nRefMechSpd] -> Data Type Conversion/1
  rss_FocController/7 -> [iActPhsCurr]
  [iActPhsCurr] -> iActPhsCurr/1
  [genXYZDutyCycl] -> rss_InverterModel/1
  [vtSplyVolt] -> rss_InverterModel/2
  [iActXYZPhsCurr] -> rss_InverterModel/3
  [tqMotTrq] -> rss_InverterModel/4
  [wActMechSpd] -> rss_InverterModel/5
  [vtXYZPhsVolt] -> rss_MotorModel/1
  [tqLoadTrq] -> rss_MotorModel/2
  [tcMagTemp] -> rss_MotorModel/3
  [tcWindTemp] -> rss_MotorModel/4
  Rate Transition9/1 -> Scope/2
  LoadTorque[Nm]/1 -> [tqManLoadTrq]
  rss_LoadModel/1 -> [tqLoadTrq]
  [tqManLoadTrq] -> rss_LoadModel/1
  [wActMechSpd] -> rss_LoadModel/2
  Constant11/1 -> Manual Switch2/1
  Constant8/1 -> Manual Switch2/2
  Manual Switch2/1 -> rss_FocController/10
  Data Type Conversion10/1 -> rss_FocController/11
  Data Type Conversion11/1 -> rss_FocController/12
  Data Type Conversion12/1 -> rss_FocController/13
  Constant14/1 -> Temperature/3(tADCMot)
  Constant13/1 -> Temperature/2(tADCPCB)
  Constant12/1 -> Temperature/1(tADCPwrTub)
  Temperature/1(tPwrTub) -> Data Type Conversion10/1
  Temperature/3(tMot) -> Data Type Conversion12/1
  Data Type Conversion1/1 -> rss_FocController/4
  rss_FocController/2 -> Terminator/1
  rss_FocController/3 -> Terminator1/1
  rss_FocController/4 -> Terminator2/1
  rss_FocController/5 -> Terminator3/1
  XYZPhaseCurrent/1(iADCXYZCurr) -> Data Type Conversion1/1
  Constant1/1 -> rss_FocController/5
  Constant5/1 -> Data Type Conversion2/1
  Data Type Conversion2/1 -> rss_FocController/6
  SupplyVoltage/1(vtADCSplyVolt) -> Data Type Conversion5/1
  Temperature/2(tPCB) -> Data Type Conversion11/1
  GDVoltage/1(vtADCtlBrdVolt) -> Data Type Conversion3/1
  [vtCtlBrdVolt] -> GDVoltage/1(vtCtlBrdVolt)
  Data Type Conversion3/1 -> rss_FocController/8
  CtlBrdVoltage[V]/1 -> [vtCtlBrdVolt]
  Data Type Conversion/1 -> sss_CommunicationCommand/1(nCommRefMechSpdRaw)
  sss_CommunicationCommand/1(nCommRefMechSpd) -> [nCommRefMechSpd]
  sss_CommunicationCommand/2(u8_modeMCUOpMode) -> [u8_modeMCUOpMode]
  [nCommRefMechSpd] -> rss_FocController/1
  [u8_modeMCUOpMode] -> rss_FocController/2
  Constant15/1 -> sss_CommunicationError/1(u8_ctLossNoDataRaw)
  sss_CommunicationError/1(u8_ctLossNoData) -> [u8_ctLossNoData]
  sss_CommunicationError/2(bol_ctComRolCnt) -> [bol_ctComRolCnt]
  [u8_ctLossNoData] -> rss_FocController/14
  [bol_ctComRolCnt] -> rss_FocController/15
  GDVoltage1/1(vtADGDVolt) -> Data Type Conversion13/1
  [vtGDVolt] -> GDVoltage1/1(vtGDVolt)
  Data Type Conversion13/1 -> rss_FocController/9
  GDVoltage[V]1/1 -> [vtGDVolt]
  Constant9/1 -> Manual Switch1/2
  Constant6/1 -> Manual Switch1/1
  Manual Switch1/1 -> rss_FocController/16
  Manual Switch3/1 -> rss_FocController/17
  Constant10/1 -> Manual Switch3/1
  Constant19/1 -> Manual Switch3/2
  Manual Switch6/1 -> rss_FocController/18
  Constant21/1 -> Manual Switch6/2
  Constant20/1 -> Manual Switch6/1
  Constant22/1 -> sss_CommunicationError/2(bol_ctComRolCntRaw)
  Constant/1 -> rss_FocController/19
  Constant26/1 -> rss_FocController/20
  Constant27/1 -> rss_FocController/21
  Constant28/1 -> rss_FocController/22
  Constant17/1 -> rss_FocController/23
  Constant23/1 -> rss_FocController/24
  Constant18/1 -> rss_FocController/25
  Constant24/1 -> rss_FocController/26
  Manual Switch5/1 -> rss_FocController/27
  Constant29/1 -> Manual Switch5/2
  Constant25/1 -> Manual Switch5/1
  Constant30/1 -> Manual Switch7/1
  Manual Switch7/1 -> rss_FocController/28
  Constant31/1 -> Manual Switch7/2
  Constant33/1 -> Manual Switch8/2
  Manual Switch8/1 -> rss_FocController/29
  Constant32/1 -> Manual Switch8/1
  Constant34/1 -> Manual Switch9/1
  Constant35/1 -> Manual Switch9/2
  Manual Switch9/1 -> rss_FocController/30
  Constant37/1 -> Manual Switch10/2
  Constant36/1 -> Manual Switch10/1
  Manual Switch10/1 -> rss_FocController/31
  Constant39/1 -> Manual Switch11/2
  Constant38/1 -> Manual Switch11/1
  Manual Switch11/1 -> rss_FocController/32
  MCUOpMode/1 -> [u8_modeMCUOpModeRaw]
  [u8_modeMCUOpModeRaw] -> Data Type Conversion9/1
  Data Type Conversion9/1 -> sss_CommunicationCommand/2(u8_modeMCUOpModeRaw)
  Constant2/1 -> rss_FocController/33
  Constant3/1 -> Manual Switch12/1
  Constant4/1 -> Manual Switch12/2
  Manual Switch12/1 -> rss_FocController/34
  Constant40/1 -> Manual Switch13/2
  Constant7/1 -> Manual Switch13/1
  Manual Switch13/1 -> rss_FocController/35
  Constant42/1 -> Manual Switch14/2
  Constant41/1 -> Manual Switch14/1
  Manual Switch14/1 -> rss_FocController/36
  Constant43/1 -> Manual Switch15/1
  Constant44/1 -> Manual Switch15/2
  Manual Switch15/1 -> rss_FocController/37
  Constant45/1 -> Data Type Conversion4/1
  Data Type Conversion4/1 -> rss_FocController/38
  rss_FocController/8 -> Terminator4/1
  rss_FocController/9 -> Terminator5/1
  Constant46/1 -> Data Type Conversion7/1
  Data Type Conversion7/1 -> rss_FocController/39
  Constant48/1 -> Manual Switch17/1
  Constant47/1 -> Manual Switch17/2
  Manual Switch17/1 -> rss_FocController/40
